simulink library "xbsIndex_r4"  (Simulink 7.1)
PreLoadFcn:
  | warning('off','MATLAB:mex:deprecatedExtension');xlmeta;com.xilinx.sysgen.util.StrategyUtil.loadAllStrategyNames();
values from neighbouring files (symbols this model uses):
  a = xpath.evaluate('//pre:DocumentInfo/pre:Document',x,javax.xml.xpath.XPathConstants.NODESET)    [xlDoc.m]
  n = xpath.evaluate(['//pre:DocumentInfo/pre:Document[@title="'  title                            '"]'],root_elem,javax.xml.xpath.XPathConstants.NODE)    [xlDoc.m]
undefined symbols (not defined in the file or in its folder): gcbh, sim_pause, simulink_period, xlBlockLoadCallback, xlipgetpartsetting, xlRegisterHandles, xlUpdateSgTokenIconStats
libraries: xbsIndex_r4 x18, xbsCopyrightNotice_r4 x1, simulink x1
(part 1 of 9)
settings Model: Tag=SysGenIndex  Creator=sysgengroup  LastModifiedBy=sysgengroup

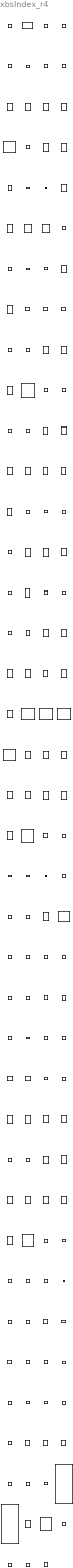
== system xbsIndex_r4 ==
  note: Xilinx Blockset v
      | (c) 2011 Xilinx, Inc.
      |
      | Library Index
  " System Generator" : Subsystem  Tag=genX  LoadFcn=xlUpdateSgTokenIconStats(gcbh);xlBlockLoadCallback(gcbh);  mask(Xilinx System Generator Block){infoedit=System Generator, xilinxfamily=Virtex6, part=xc6vsx315t, speed=-3, package=ff1156, synthesis_tool_sgadvanced=, synthesis_tool=XST, clock_wrapper_sgadvanced=, clock_wrapper=Clock Enables, directory=./netlist, proj_type_sgadvanced=, proj_type=Project Navigator, Synth_file_sgadvanced=, Synth_file=XST Defaults, Impl_file_sgadvanced=, Impl_file=ISE Defaults, testbench_sgadvanced=, testbench=off, simulink_period=1, sysclk_period=10, dcm_input_clock_period=10, incr_netlist_sgadvanced=, incr_netlist=off, trim_vbits_sgadvanced=, trim_vbits=Everywhere in SubSystem, dbl_ovrd_sgadvanced=, dbl_ovrd=According to Block Masks, core_generation_sgadvanced=, core_generation=According to Block Masks, run_coregen_sgadvanced=, run_coregen=off, deprecated_control_sgadvanced=, deprecated_control=off, eval_field=0, has_advanced_control=0, sggui_pos=-1,-1,-1,-1, block_type=sysgen, block_version=, sg_icon_stat=50,50,-1,-1,token,white,0,07734,right,,[ ],[ ], sg_mask_display=|, sg_list_contents=, sg_blockgui_xml=}
      mask sg_mask_display=|
      | fprintf('','COMMENT: begin icon graphics');
      | patch([0 50 50 0 0 ],[0 0 50 50 0 ],[1 1 1 ]);
      | patch([1.6375 16.81 27.31 37.81 48.31 27.31 12.1375 1.6375 ],[36.655 36.655 47.155 36.655 47.155 47.155 47.155 36.655 ],[0.933333 0.203922 0.141176 ]);
      | patch([12.1375 27.31 16.81 1.6375 12.1375 ],[26.155 26.155 36.655 36.655 26.155 ],[0.698039 0.0313725 0.219608 ]);
      | patch([1.6375 16.81 27.31 12.1375 1.6375 ],[15.655 15.655 26.155 26.155 15.655 ],[0.933333 0.203922 0.141176 ]);
      | patch([12.1375 48.31 37.81 27.31 16.81 1.6375 12.1375 ],[5.155 5.155 15.655 5.155 15.655 15.655 5.155 ],[0.698039 0.0313725 0.219608 ]);
      | fprintf('','COMMENT: end icon graphics');
      | fprintf('','COMMENT: begin icon text');
      | fprintf('','COMMENT: end icon text');
      mask prompts: infoedit ""; xilinxfamily "Xilinx family"; synthesis_tool_sgadvanced ""; synthesis_tool "Synthesis tool"; clock_wrapper_sgadvanced ""; clock_wrapper "Clock Wrapper"; directory "Target directory"; proj_type_sgadvanced ""; proj_type "Project Type"; Synth_file_sgadvanced ""; Synth_file "Synthesis strategy"; Impl_file_sgadvanced ""; Impl_file "Implementation strategy"; testbench_sgadvanced ""; simulink_period "Simulink period"; sysclk_period "System clock period"; dcm_input_clock_period "DCM input clock period"; incr_netlist_sgadvanced ""; incr_netlist "Incremental netlisting"; trim_vbits_sgadvanced ""; trim_vbits "Trim valid bits"; dbl_ovrd_sgadvanced ""; dbl_ovrd "Override with doubles"; core_generation_sgadvanced ""; core_generation "Generate cores"; run_coregen_sgadvanced ""; run_coregen "Run CoreGen"; deprecated_control_sgadvanced ""; deprecated_control "Show deprecated controls"; eval_field ""; has_advanced_control ""; sggui_pos ""; block_type ""; block_version ""; sg_icon_stat ""; sg_mask_display ""; sg_list_contents ""; sg_blockgui_xml ""
      mask help: System Generator
      mask init:
      | try
      |   tmp_gcb = gcb;
      |   tmp_gcbh = gcbh;
      |   if (strcmp('SysGenIndex',get_param(bdroot(tmp_gcbh),'tag')) && ~isempty(regexp(bdroot(tmp_gcb), '^xbs', 'once')))
      |     return;
      |   end;
      |   xlMungeMaskParams;
      | 
      |   block_type='sysgen';
      | 
      |   serialized_declarations = '{''block_type''=>''String''}';
      |   ptable_ = xlblockprep(get_param(tmp_gcb, 'MaskWSVariables'));
      |   try
      |     xlBlockMoveCallback(tmp_gcbh);
      |   catch 
      |      clear global xl_updateicon_recursion_guard;
      |   end;
      | catch
      |   global dbgsysgen;
      |   if(~isempty(dbgsysgen) && dbgsysgen)
      |     e = regexprep(lasterr, '\n', '\nError: ');
      |     disp(['Error: While running MaskInit code on block ' tmp_gcb ': ' e]);
      |     error(e);
      |   end
      | end
      settings: AttributesFormatString=System\nGenerator  CopyFcn=xlBlockMoveCallback(gcbh);  DeleteFcn=xlSysgenGUI('delete', gcs, gcbh);  ModelCloseFcn=xlSysgenGUI('Close',gcs,gcbh);  PostSaveFcn=xlSysgenGUI('Save')  OpenFcn=xlSysgenGUI('startup',gcs,gcbh);  MoveFcn=xlBlockMoveCallback(gcbh);
      mask Help: eval('');xlDoc('-book','sysgen','-topic','System_Generator');
      mask StyleString: edit,edit,edit,edit,edit,edit,popup(Spectrum|Synplify|Synplify Pro|XST|RDS|Precision),edit,popup(Clock Enables|Clock Generator(DCM)|Expose Clock Ports),edit,edit,popup(Project Navigator|PlanAhead),edit,popup(XST Defaults|PlanAhead Defaults|Rodin Synthesis Defaults),edit,popup(ISE Defaults|Rodin Implementation Defaults),edit,checkbox,edit,edit,edit,edit,checkbox,edit,popup(According to Block Masks|Everywhere in SubSystem|No Where in SubSystem),edit,popup(According to Block Masks|Everywhere in SubSystem|No Where in SubSystem),edit,popup(According to Block Masks|Everywhere Available|Not Needed - Already Generated),edit,checkbox,edit,checkbox,edit,edit,edit,edit,edit,edit,edit,edit,edit
      mask Display:
      | fprintf('','COMMENT: begin icon graphics');
      | patch([0 50 50 0 0 ],[0 0 50 50 0 ],[1 1 1 ]);
      | patch([1.6375 16.81 27.31 37.81 48.31 27.31 12.1375 1.6375 ],[36.655 36.655 47.155 36.655 47.155 47.155 47.155 36.655 ],[0.933333 0.203922 0.141176 ]);
      | patch([12.1375 27.31 16.81 1.6375 12.1375 ],[26.155 26.155 36.655 36.655 26.155 ],[0.698039 0.0313725 0.219608 ]);
      | patch([1.6375 16.81 27.31 12.1375 1.6375 ],[15.655 15.655 26.155 26.155 15.655 ],[0.933333 0.203922 0.141176 ]);
      | patch([12.1375 48.31 37.81 27.31 16.81 1.6375 12.1375 ],[5.155 5.155 15.655 5.155 15.655 15.655 5.155 ],[0.698039 0.0313725 0.219608 ]);
      | fprintf('','COMMENT: end icon graphics');
      | fprintf('','COMMENT: begin icon text');
      | fprintf('','COMMENT: end icon text');
  AXI FIFO : S-Function  LoadFcn=xlBlockLoadCallback(gcbh);  FunctionName=sysgen  Parameters=ptable_  EnableBusSupport=off  mask(Xilinx AXI FIFO Block Block){input_depth_axis_sgadvanced=, input_depth_axis=1K, actual_fifo_depth_label=1026, enable_tdata_sgadvanced=, enable_tdata=on, enable_tdest_sgadvanced=, enable_tdest=off, enable_tstrb_sgadvanced=, enable_tstrb=off, enable_tready_sgadvanced=, enable_tready=on, enable_tid_sgadvanced=, enable_tid=off, enable_tuser_sgadvanced=, enable_tuser=off, enable_tkeep_sgadvanced=, enable_tkeep=off, enable_tlast_sgadvanced=, enable_tlast=off, has_aresetn_sgadvanced=, has_aresetn=off, underflow_flag_axi_sgadvanced=, underflow_flag_axi=off, underflow_sense_axi_sgadvanced=, underflow_sense_axi=Active High, overflow_flag_axi_sgadvanced=, overflow_flag_axi=off, overflow_sense_axi_sgadvanced=, overflow_sense_axi=Active High, enable_data_counts_axis_sgadvanced=, enable_data_counts_axis=off, fifo_implementation_type_axis_sgadvanced=, fifo_implementation_type_axis=Common Clock Block RAM, trim_axipin_name=on, xlcconfig=, programmable_full_type_axis=Full, full_threshold_assert_value_axis=0, programmable_empty_type_axis=Empty, empty_threshold_assert_value_axis=1022, has_advanced_control=0, sggui_pos=-1,-1,-1,-1, block_type=axi_fifo, block_version=, sg_icon_stat=200,114,3,3,white,blue,0,6408c73b,right,,[2 3 3 ],[2 2 3 ], sg_mask_display=|, sg_list_contents=, sg_blockgui_xml=}
      mask sg_mask_display=|
      | fprintf('','COMMENT: begin icon graphics');
      | patch([0 0 4 4 ],[111 83 83 111 ],[5.466667e-001 5.800000e-001 6.400000e-001 ]);
      | patch([0 0 4 4 ],[71 3 3 71 ],[3.233333e-001 3.400000e-001 3.700000e-001 ]);
      | patch([196 196 200 200 ],[111 43 43 111 ],[5.466667e-001 5.800000e-001 6.400000e-001 ]);
      | patch([196 196 200 200 ],[31 3 3 31 ],[3.233333e-001 3.400000e-001 3.700000e-001 ]);
      | patch([4 195 195 4 4 ],[0 0 114 114 0 ],[7.700000e-001 8.200000e-001 9.100000e-001 ]);
      | plot([4 195 195 4 4 ],[0 0 114 114 0 ]);
      |
      |
      | patch([64.4 87.52 103.52 119.52 135.52 103.52 80.4 64.4 ],[74.76 74.76 90.76 74.76 90.76 90.76 90.76 74.76 ],[1 1 1 ]);
      | patch([80.4 103.52 87.52 64.4 80.4 ],[58.76 58.76 74.76 74.76 58.76 ],[0.931 0.946 0.973 ]);
      | patch([64.4 87.52 103.52 80.4 64.4 ],[42.76 42.76 58.76 58.76 42.76 ],[1 1 1 ]);
      | patch([80.4 135.52 119.52 103.52 87.52 64.4 80.4 ],[26.76 26.76 42.76 26.76 42.76 42.76 26.76 ],[0.931 0.946 0.973 ]);
      | fprintf('','COMMENT: end icon graphics');
      | fprintf('','COMMENT: begin icon text');
      | color('black');port_label('input',1,'  tready  ');
      | color('black');port_label('input',2,'  tvalid  ');
      | color('black');port_label('input',3,'  tdata  ');
      | color('black');port_label('output',1,'  tvalid  ');
      | color('black');port_label('output',2,'  tdata  ');
      | color('black');port_label('output',3,'  tready  ');
      | fprintf('','COMMENT: end icon text');
      mask prompts: input_depth_axis_sgadvanced ""; input_depth_axis "FIFO depth"; actual_fifo_depth_label "Actual FIFO depth"; enable_tdata_sgadvanced ""; enable_tdata "TDATA"; enable_tdest_sgadvanced ""; enable_tdest "TDEST"; enable_tstrb_sgadvanced ""; enable_tstrb "TSTRB"; enable_tready_sgadvanced ""; enable_tready "TREADY"; enable_tid_sgadvanced ""; enable_tid "TID"; enable_tuser_sgadvanced ""; enable_tuser "TUSER"; enable_tkeep_sgadvanced ""; enable_tkeep "TKEEP"; enable_tlast_sgadvanced ""; enable_tlast "TLAST"; has_aresetn_sgadvanced ""; has_aresetn "aresetn"; underflow_flag_axi_sgadvanced ""; underflow_flag_axi "Underflow flag"; underflow_sense_axi_sgadvanced ""; underflow_sense_axi "Underflow (Read Error)"; overflow_flag_axi_sgadvanced ""; overflow_flag_axi "Overflow flag"; overflow_sense_axi_sgadvanced ""; overflow_sense_axi "Overflow (Read Error)"; enable_data_counts_axis_sgadvanced ""; enable_data_counts_axis "Provide FIFO occupancy DATA counts"; fifo_implementation_type_axis_sgadvanced ""; fifo_implementation_type_axis "FIFO implementation type"; trim_axipin_name "Display shortened port names"; xlcconfig ""; programmable_full_type_axis ""; full_threshold_assert_value_axis ""; programmable_empty_type_axis ""; empty_threshold_assert_value_axis ""; has_advanced_control ""; sggui_pos ""; block_type ""; block_version ""; sg_icon_stat ""; sg_mask_display ""; sg_list_contents ""; sg_blockgui_xml ""
      mask help: Xilinx AXI FIFO Block
      mask init:
      | try
      |   tmp_gcb = gcb;
      |   tmp_gcbh = gcbh;
      |   if (strcmp('SysGenIndex',get_param(bdroot(tmp_gcbh),'tag')) && ~isempty(regexp(bdroot(tmp_gcb), '^xbs', 'once')))
      |     return;
      |   end;
      |   xlMungeMaskParams;
      |   block_config = 'sysgen_blockset:AXI_FIFO_config';
      | 
      |   block_type='axi_fifo';
      | 
      |   serialized_declarations = '{''actual_fifo_depth_label''=>''Int'',''empty_threshold_assert_value_axis''=>''Int'',''enable_data_counts_axis''=>''Bool'',''enable_tdata''=>''Bool'',''enable_tdest''=>''Bool'',''enable_tid''=>''Bool'',''enable_tkeep''=>''Bool'',''enable_tlast''=>''Bool'',''enable_tready''=>''Bool'',''enable_tstrb''=>''Bool'',''enable_tuser''=>''Bool'',''fifo_implementation_type_axis''=>''String'',''full_threshold_assert_value_axis''=>''Int'',''has_aresetn''=>''Bool'',''input_depth_axis''=>''Int'',''overflow_flag_axi''=>''Bool'',''overflow_sense_axi''=>''String'',''programmable_empty_type_axis''=>''String'',''programmable_full_type_axis''=>''String'',''trim_axipin_name''=>''Int'',''underflow_flag_axi''=>''Bool'',''underflow_sense_axi''=>''String'',''xlcconfig''=>''String'',''block_type''=>''String''}';
      |   ptable_ = xlblockprep(get_param(tmp_gcb, 'MaskWSVariables'));
      |   try
      |     xlBlockMoveCallback(tmp_gcbh);
      |   catch 
      |      clear global xl_updateicon_recursion_guard;
      |   end;
      | catch
      |   global dbgsysgen;
      |   if(~isempty(dbgsysgen) && dbgsysgen)
      |     e = regexprep(lasterr, '\n', '\nError: ');
      |     disp(['Error: While running MaskInit code on block ' tmp_gcb ': ' e]);
      |     error(e);
      |   end
      | end
      settings: CopyFcn=xlBlockMoveCallback(gcbh);  DeleteFcn=xlDestroyGui(gcbh);  ModelCloseFcn=xlDestroyGui(gcbh);  PreSaveFcn=xlBlockPreSaveCallback(gcbh);  PostSaveFcn=xlBlockPostSaveCallback(gcbh);  DestroyFcn=xlDestroyGui(gcbh);  OpenFcn=xlOpenGui(gcbh, 'axi_fifo_gui.xml', @axi_fifo_enablement, @axi_fifo_action)  CloseFcn=xlDestroyGui(gcbh);  MoveFcn=xlBlockMoveCallback(gcbh);
      mask Help: eval('');xlDoc('-book','sysgen','-topic','AXI_FIFO');
      mask StyleString: edit,popup(16|32|64|128|256|512|1K|2K|4K|8K|16K|32K|64K|128K|256K|512K|1M|2M|4M),edit,edit,checkbox,edit,checkbox,edit,checkbox,edit,checkbox,edit,checkbox,edit,checkbox,edit,checkbox,edit,checkbox,edit,checkbox,edit,checkbox,edit,popup(Active High|Active Low),edit,checkbox,edit,popup(Active High|Active Low),edit,checkbox,edit,popup(Common Clock Block RAM|Common Clock Distributed RAM),checkbox,edit,edit,edit,edit,edit,edit,edit,edit,edit,edit,edit,edit,edit
      mask Display:
      | fprintf('','COMMENT: begin icon graphics');
      | patch([0 0 4 4 ],[111 83 83 111 ],[5.466667e-001 5.800000e-001 6.400000e-001 ]);
      | patch([0 0 4 4 ],[71 3 3 71 ],[3.233333e-001 3.400000e-001 3.700000e-001 ]);
      | patch([196 196 200 200 ],[111 43 43 111 ],[5.466667e-001 5.800000e-001 6.400000e-001 ]);
      | patch([196 196 200 200 ],[31 3 3 31 ],[3.233333e-001 3.400000e-001 3.700000e-001 ]);
      | patch([4 195 195 4 4 ],[0 0 114 114 0 ],[7.700000e-001 8.200000e-001 9.100000e-001 ]);
      | plot([4 195 195 4 4 ],[0 0 114 114 0 ]);
      | 
      | 
      | patch([64.4 87.52 103.52 119.52 135.52 103.52 80.4 64.4 ],[74.76 74.76 90.76 74.76 90.76 90.76 90.76 74.76 ],[1 1 1 ]);
      | patch([80.4 103.52 87.52 64.4 80.4 ],[58.76 58.76 74.76 74.76 58.76 ],[0.931 0.946 0.973 ]);
      | patch([64.4 87.52 103.52 80.4 64.4 ],[42.76 42.76 58.76 58.76 42.76 ],[1 1 1 ]);
      | patch([80.4 135.52 119.52 103.52 87.52 64.4 80.4 ],[26.76 26.76 42.76 26.76 42.76 42.76 26.76 ],[0.931 0.946 0.973 ]);
      | fprintf('','COMMENT: end icon graphics');
      | fprintf('','COMMENT: begin icon text');
      | color('black');port_label('input',1,'  tready  ');
      | color('black');port_label('input',2,'  tvalid  ');
      | color('black');port_label('input',3,'  tdata  ');
      | color('black');port_label('output',1,'  tvalid  ');
      | color('black');port_label('output',2,'  tdata  ');
      | color('black');port_label('output',3,'  tready  ');
      | fprintf('','COMMENT: end icon text');
  Accumulator : S-Function  LoadFcn=xlBlockLoadCallback(gcbh);  FunctionName=sysgen  Parameters=ptable_  EnableBusSupport=off  mask(Xilinx Accumulator Block){infoedit=Adder or subtracter-based accumulator.   Output type and binary point position match the input.<br><br>Hardware notes: When "Reinitialize with input 'b' on reset" is selected, the accumulator is forced to run at the system rate even if the input 'b' is running at a slower rate., operation_sgadvanced=, operation=Add, n_bits=8, overflow_sgadvanced=, overflow=Wrap, scale_sgadvanced=, scale=1, rst_sgadvanced=, rst=on, hasbypass_sgadvanced=, hasbypass=off, en_sgadvanced=, en=off, dbl_ovrd_sgadvanced=, dbl_ovrd=off, use_behavioral_HDL_sgadvanced=, use_behavioral_HDL=on, implementation_sgadvanced=, implementation=Fabric, xl_use_area_sgadvanced=, xl_use_area=off, xl_area=[0,0,0,0,0,0,0], has_advanced_control=0, sggui_pos=-1,-1,-1,-1, block_type=accum, block_version=, sg_icon_stat=60,58,2,1,white,blue,0,6949434e,right,,[ ],[ ], sg_mask_display=|, sg_list_contents=, sg_blockgui_xml=}
      mask sg_mask_display=|
      | fprintf('','COMMENT: begin icon graphics');
      | patch([0 60 60 0 0 ],[0 0 58 58 0 ],[0.77 0.82 0.91 ]);
      | plot([0 60 60 0 0 ],[0 0 58 58 0 ]);
      | patch([12.2 23.76 31.76 39.76 47.76 31.76 20.2 12.2 ],[37.88 37.88 45.88 37.88 45.88 45.88 45.88 37.88 ],[1 1 1 ]);
      | patch([20.2 31.76 23.76 12.2 20.2 ],[29.88 29.88 37.88 37.88 29.88 ],[0.931 0.946 0.973 ]);
      | patch([12.2 23.76 31.76 20.2 12.2 ],[21.88 21.88 29.88 29.88 21.88 ],[1 1 1 ]);
      | patch([20.2 47.76 39.76 31.76 23.76 12.2 20.2 ],[13.88 13.88 21.88 13.88 21.88 21.88 13.88 ],[0.931 0.946 0.973 ]);
      | fprintf('','COMMENT: end icon graphics');
      | fprintf('','COMMENT: begin icon text');
      | color('black');port_label('input',1,'b');
      | color('black');port_label('input',2,'rst');
      | color('black');port_label('output',1,'\bf+=b','texmode','on');
      | fprintf('','COMMENT: end icon text');
      mask prompts: infoedit ""; operation_sgadvanced ""; n_bits "Number of bits"; overflow_sgadvanced ""; scale_sgadvanced ""; scale "Feedback scaling"; rst_sgadvanced ""; rst "Provide synchronous reset port"; hasbypass_sgadvanced ""; hasbypass "Reinitialize with input 'b' on reset"; en_sgadvanced ""; en "Provide enable port"; dbl_ovrd_sgadvanced ""; dbl_ovrd "Override with doubles"; use_behavioral_HDL_sgadvanced ""; use_behavioral_HDL "Use behavioral HDL (otherwise use core)"; implementation_sgadvanced ""; implementation "Implement using"; xl_use_area_sgadvanced ""; xl_use_area "Define FPGA area for resource estimation"; xl_area "FPGA area [slices, FFs, BRAMs, LUTs, IOBs, emb. mults, TBUFs]"; has_advanced_control ""; sggui_pos ""; block_type ""; block_version ""; sg_icon_stat ""; sg_mask_display ""; sg_list_contents ""; sg_blockgui_xml ""
      mask help:
      | Adder or subtracter-based accumulator.   Output type and binary point position match the input.
      |
      | Hardware notes: When "Reinitialize with input 'b' on reset" is selected, the accumulator is forced to run at the system rate even if the input 'b' is running at a slower rate.
      mask init:
      | try
      |   tmp_gcb = gcb;
      |   tmp_gcbh = gcbh;
      |   if (strcmp('SysGenIndex',get_param(bdroot(tmp_gcbh),'tag')) && ~isempty(regexp(bdroot(tmp_gcb), '^xbs', 'once')))
      |     return;
      |   end;
      |   xlMungeMaskParams;
      |   block_config = 'sysgen_blockset:Accum_config';
      | 
      |   block_type='accum';
      | 
      |   serialized_declarations = '{''en''=>''Int'',''hasbypass''=>''Int'',''implementation''=>''String'',''n_bits''=>''Int'',''operation''=>''Int'',''overflow''=>''Int'',''rst''=>''Int'',''scale''=>''Int'',''use_behavioral_HDL''=>''Int'',''block_type''=>''String''}';
      |   ptable_ = xlblockprep(get_param(tmp_gcb, 'MaskWSVariables'));
      |   try
      |     xlBlockMoveCallback(tmp_gcbh);
      |   catch 
      |      clear global xl_updateicon_recursion_guard;
      |   end;
      | catch
      |   global dbgsysgen;
      |   if(~isempty(dbgsysgen) && dbgsysgen)
      |     e = regexprep(lasterr, '\n', '\nError: ');
      |     disp(['Error: While running MaskInit code on block ' tmp_gcb ': ' e]);
      |     error(e);
      |   end
      | end
      settings: CopyFcn=xlBlockMoveCallback(gcbh);  DeleteFcn=xlDestroyGui(gcbh);  ModelCloseFcn=xlDestroyGui(gcbh);  PreSaveFcn=xlBlockPreSaveCallback(gcbh);  PostSaveFcn=xlBlockPostSaveCallback(gcbh);  DestroyFcn=xlDestroyGui(gcbh);  OpenFcn=xlOpenGui(gcbh, 'accum_gui.xml', @accumenablement, -1)  CloseFcn=xlDestroyGui(gcbh);  MoveFcn=xlBlockMoveCallback(gcbh);
      mask Help: eval('');xlDoc('-book','sysgen','-topic','Accumulator');
      mask StyleString: edit,edit,popup(Add|Subtract),edit,edit,popup(Wrap|Saturate|Flag as error),edit,popup(1|1/2|1/4|1/8|1/16|1/32|1/64|1/128|1/256),edit,checkbox,edit,checkbox,edit,checkbox,edit,checkbox,edit,checkbox,edit,popup(Fabric|DSP48),edit,checkbox,edit,edit,edit,edit,edit,edit,edit,edit,edit
      mask Display:
      | fprintf('','COMMENT: begin icon graphics');
      | patch([0 60 60 0 0 ],[0 0 58 58 0 ],[0.77 0.82 0.91 ]);
      | plot([0 60 60 0 0 ],[0 0 58 58 0 ]);
      | patch([12.2 23.76 31.76 39.76 47.76 31.76 20.2 12.2 ],[37.88 37.88 45.88 37.88 45.88 45.88 45.88 37.88 ],[1 1 1 ]);
      | patch([20.2 31.76 23.76 12.2 20.2 ],[29.88 29.88 37.88 37.88 29.88 ],[0.931 0.946 0.973 ]);
      | patch([12.2 23.76 31.76 20.2 12.2 ],[21.88 21.88 29.88 29.88 21.88 ],[1 1 1 ]);
      | patch([20.2 47.76 39.76 31.76 23.76 12.2 20.2 ],[13.88 13.88 21.88 13.88 21.88 21.88 13.88 ],[0.931 0.946 0.973 ]);
      | fprintf('','COMMENT: end icon graphics');
      | fprintf('','COMMENT: begin icon text');
      | color('black');port_label('input',1,'b');
      | color('black');port_label('input',2,'rst');
      | color('black');port_label('output',1,'\bf+=b','texmode','on');
      | fprintf('','COMMENT: end icon text');
  AddSub : S-Function  LoadFcn=xlBlockLoadCallback(gcbh);  FunctionName=sysgen  Parameters=ptable_  EnableBusSupport=off  mask(Xilinx Adder/Subtracter Block){mode_sgadvanced=, mode=Addition, use_carryin_sgadvanced=, use_carryin=off, use_carryout_sgadvanced=, use_carryout=off, en_sgadvanced=, en=off, latency=0, precision_sgadvanced=, precision=Full, arith_type_sgadvanced=, arith_type=Unsigned, n_bits=16, bin_pt=14, quantization_sgadvanced=, quantization=Truncate, overflow_sgadvanced=, overflow=Wrap, dbl_ovrd_sgadvanced=, dbl_ovrd=off, use_behavioral_HDL_sgadvanced=, use_behavioral_HDL=off, hw_selection_sgadvanced=, hw_selection=Fabric, pipelined_sgadvanced=, pipelined=off, xl_use_area_sgadvanced=, xl_use_area=off, xl_area=[0,0,0,0,0,0,0], use_rpm=, has_advanced_control=0, sggui_pos=-1,-1,-1,-1, block_type=addsub, block_version=, sg_icon_stat=60,58,2,1,white,blue,0,e139daf6,right,,[ ],[ ], sg_mask_display=|, sg_list_contents=, sg_blockgui_xml=}
      mask sg_mask_display=|
      | fprintf('','COMMENT: begin icon graphics');
      | patch([0 60 60 0 0 ],[0 0 58 58 0 ],[0.77 0.82 0.91 ]);
      | plot([0 60 60 0 0 ],[0 0 58 58 0 ]);
      | patch([12.2 23.76 31.76 39.76 47.76 31.76 20.2 12.2 ],[37.88 37.88 45.88 37.88 45.88 45.88 45.88 37.88 ],[1 1 1 ]);
      | patch([20.2 31.76 23.76 12.2 20.2 ],[29.88 29.88 37.88 37.88 29.88 ],[0.931 0.946 0.973 ]);
      | patch([12.2 23.76 31.76 20.2 12.2 ],[21.88 21.88 29.88 29.88 21.88 ],[1 1 1 ]);
      | patch([20.2 47.76 39.76 31.76 23.76 12.2 20.2 ],[13.88 13.88 21.88 13.88 21.88 21.88 13.88 ],[0.931 0.946 0.973 ]);
      | fprintf('','COMMENT: end icon graphics');
      | fprintf('','COMMENT: begin icon text');
      | color('black');port_label('input',1,'a');
      | color('black');port_label('input',2,'b');
      | color('black');port_label('output',1,'\bf{a + b}','texmode','on');
      | fprintf('','COMMENT: end icon text');
      mask prompts: mode_sgadvanced ""; mode "Operation"; use_carryin_sgadvanced ""; use_carryin "Provide carry-in port"; use_carryout_sgadvanced ""; use_carryout "Provide carry-out port"; en_sgadvanced ""; en "Provide enable port"; precision_sgadvanced ""; arith_type_sgadvanced ""; arith_type "Arithmetic type"; n_bits "Number of bits"; bin_pt "Binary point"; quantization_sgadvanced ""; overflow_sgadvanced ""; dbl_ovrd_sgadvanced ""; dbl_ovrd "Override with doubles"; use_behavioral_HDL_sgadvanced ""; use_behavioral_HDL "Use behavioral HDL (otherwise use core)"; hw_selection_sgadvanced ""; hw_selection "Implement using"; pipelined_sgadvanced ""; pipelined "Pipeline for maximum performance"; xl_use_area_sgadvanced ""; xl_use_area "Define FPGA area for resource estimation"; xl_area "FPGA area [slices, FFs, BRAMs, LUTs, IOBs, emb. mults, TBUFs]"; use_rpm ""; has_advanced_control ""; sggui_pos ""; block_type ""; block_version ""; sg_icon_stat ""; sg_mask_display ""; sg_list_contents ""; sg_blockgui_xml ""
      mask help: Xilinx Adder/Subtracter
      mask init:
      | try
      |   tmp_gcb = gcb;
      |   tmp_gcbh = gcbh;
      |   if (strcmp('SysGenIndex',get_param(bdroot(tmp_gcbh),'tag')) && ~isempty(regexp(bdroot(tmp_gcb), '^xbs', 'once')))
      |     return;
      |   end;
      |   xlMungeMaskParams;
      |   block_config = 'sysgen_blockset:Addsub_config';
      | 
      |   block_type='addsub';
      | 
      |   serialized_declarations = '{''arith_type''=>''Int'',''bin_pt''=>''Int'',''en''=>''Int'',''hw_selection''=>''String'',''latency''=>''Int'',''mode''=>''Int'',''n_bits''=>''Int'',''overflow''=>''Int'',''pipelined''=>''Int'',''precision''=>''Int'',''quantization''=>''Int'',''rst''=>''Int'',''use_behavioral_HDL''=>''Int'',''use_carryin''=>''Int'',''use_carryout''=>''Int'',''use_rpm''=>''String'',''block_type''=>''String''}';
      |   ptable_ = xlblockprep(get_param(tmp_gcb, 'MaskWSVariables'));
      |   try
      |     xlBlockMoveCallback(tmp_gcbh);
      |   catch 
      |      clear global xl_updateicon_recursion_guard;
      |   end;
      | catch
      |   global dbgsysgen;
      |   if(~isempty(dbgsysgen) && dbgsysgen)
      |     e = regexprep(lasterr, '\n', '\nError: ');
      |     disp(['Error: While running MaskInit code on block ' tmp_gcb ': ' e]);
      |     error(e);
      |   end
      | end
      settings: CopyFcn=xlBlockMoveCallback(gcbh);  DeleteFcn=xlDestroyGui(gcbh);  ModelCloseFcn=xlDestroyGui(gcbh);  PreSaveFcn=xlBlockPreSaveCallback(gcbh);  PostSaveFcn=xlBlockPostSaveCallback(gcbh);  DestroyFcn=xlDestroyGui(gcbh);  OpenFcn=xlOpenGui(gcbh, 'addsub_gui.xml', @addsubenablement, -1)  CloseFcn=xlDestroyGui(gcbh);  MoveFcn=xlBlockMoveCallback(gcbh);
      mask Help: eval('');xlDoc('-book','sysgen','-topic','AddSub');
      mask StyleString: edit,popup(Addition|Subtraction|Addition or Subtraction),edit,checkbox,edit,checkbox,edit,checkbox,edit,edit,popup(Full|User Defined),edit,popup(Signed  (2's comp)|Unsigned),edit,edit,edit,popup(Truncate|Round  (unbiased: +/- Inf)),edit,popup(Wrap|Saturate|Flag as error),edit,checkbox,edit,checkbox,edit,popup(Fabric|DSP48),edit,checkbox,edit,checkbox,edit,edit,edit,edit,edit,edit,edit,edit,edit,edit
      mask Display:
      | fprintf('','COMMENT: begin icon graphics');
      | patch([0 60 60 0 0 ],[0 0 58 58 0 ],[0.77 0.82 0.91 ]);
      | plot([0 60 60 0 0 ],[0 0 58 58 0 ]);
      | patch([12.2 23.76 31.76 39.76 47.76 31.76 20.2 12.2 ],[37.88 37.88 45.88 37.88 45.88 45.88 45.88 37.88 ],[1 1 1 ]);
      | patch([20.2 31.76 23.76 12.2 20.2 ],[29.88 29.88 37.88 37.88 29.88 ],[0.931 0.946 0.973 ]);
      | patch([12.2 23.76 31.76 20.2 12.2 ],[21.88 21.88 29.88 29.88 21.88 ],[1 1 1 ]);
      | patch([20.2 47.76 39.76 31.76 23.76 12.2 20.2 ],[13.88 13.88 21.88 13.88 21.88 21.88 13.88 ],[0.931 0.946 0.973 ]);
      | fprintf('','COMMENT: end icon graphics');
      | fprintf('','COMMENT: begin icon text');
      | color('black');port_label('input',1,'a');
      | color('black');port_label('input',2,'b');
      | color('black');port_label('output',1,'\bf{a + b}','texmode','on');
      | fprintf('','COMMENT: end icon text');
  Addressable Shift Register : S-Function  LoadFcn=xlBlockLoadCallback(gcbh);  FunctionName=sysgen  Parameters=ptable_  EnableBusSupport=off  mask(Xilinx Addressable Shift Register Block){infoedit=Delay of configurable length.  Any element in the delay line can be addressed and driven onto the output port.<br><br>Hardware notes: This block is implemented using SRL16s. If Virtex-4 or Spartan-3 device is used, multiple SRLC16s are cascaded together., infer_latency_sgadvanced=, infer_latency=off, depth=2, initVector=[0], en_sgadvanced=, en=off, dbl_ovrd_sgadvanced=, dbl_ovrd=off, use_behavioral_HDL_sgadvanced=, use_behavioral_HDL=off, Optimization_sgadvanced=, Optimization=Resource, xl_use_area_sgadvanced=, xl_use_area=off, xl_area=[0,0,0,0,0,0,0], use_rpm=, xlcconfig=, has_advanced_control=0, sggui_pos=-1,-1,-1,-1, block_type=addrsr, block_version=, sg_icon_stat=60,58,2,1,white,blue,0,a352fb33,right,,[ ],[ ], sg_mask_display=|, sg_list_contents=, sg_blockgui_xml=}
      mask sg_mask_display=|
      | fprintf('','COMMENT: begin icon graphics');
      | patch([0 60 60 0 0 ],[0 0 58 58 0 ],[0.77 0.82 0.91 ]);
      | plot([0 60 60 0 0 ],[0 0 58 58 0 ]);
      | patch([12.2 23.76 31.76 39.76 47.76 31.76 20.2 12.2 ],[37.88 37.88 45.88 37.88 45.88 45.88 45.88 37.88 ],[1 1 1 ]);
      | patch([20.2 31.76 23.76 12.2 20.2 ],[29.88 29.88 37.88 37.88 29.88 ],[0.931 0.946 0.973 ]);
      | patch([12.2 23.76 31.76 20.2 12.2 ],[21.88 21.88 29.88 29.88 21.88 ],[1 1 1 ]);
      | patch([20.2 47.76 39.76 31.76 23.76 12.2 20.2 ],[13.88 13.88 21.88 13.88 21.88 21.88 13.88 ],[0.931 0.946 0.973 ]);
      | fprintf('','COMMENT: end icon graphics');
      | fprintf('','COMMENT: begin icon text');
      | color('black');port_label('input',1,'d');
      | color('black');port_label('input',2,'addr');
      | color('black');port_label('output',1,'q');
      | fprintf('','COMMENT: end icon text');
      mask prompts: infoedit ""; infer_latency_sgadvanced ""; infer_latency "Infer maximum latency (depth) using address port width"; depth "Maximum latency (depth)"; initVector "Initial value vector"; en_sgadvanced ""; en "Provide enable port"; dbl_ovrd_sgadvanced ""; dbl_ovrd "Override with doubles"; use_behavioral_HDL_sgadvanced ""; use_behavioral_HDL "Use behavioral HDL (otherwise use core)"; Optimization_sgadvanced ""; xl_use_area_sgadvanced ""; xl_use_area "Define FPGA area for resource estimation"; xl_area "FPGA area [slices, FFs, BRAMs, LUTs, IOBs, emb. mults, TBUFs]"; use_rpm ""; xlcconfig ""; has_advanced_control ""; sggui_pos ""; block_type ""; block_version ""; sg_icon_stat ""; sg_mask_display ""; sg_list_contents ""; sg_blockgui_xml ""
      mask help:
      | Delay of configurable length.  Any element in the delay line can be addressed and driven onto the output port.
      |
      | Hardware notes: This block is implemented using SRL16s. If Virtex-4 or Spartan-3 device is used, multiple SRLC16s are cascaded together.
      mask init:
      | try
      |   tmp_gcb = gcb;
      |   tmp_gcbh = gcbh;
      |   if (strcmp('SysGenIndex',get_param(bdroot(tmp_gcbh),'tag')) && ~isempty(regexp(bdroot(tmp_gcb), '^xbs', 'once')))
      |     return;
      |   end;
      |   xlMungeMaskParams;
      |   block_config = 'sysgen_blockset:Addrsr_config';
      | 
      |   block_type='addrsr';
      | 
      |   serialized_declarations = '{''Optimization''=>''Int'',''depth''=>''Int'',''en''=>''Int'',''infer_latency''=>''Int'',''initVector''=>''DoubleVector'',''rpm''=>''Int'',''rst''=>''Int'',''use_behavioral_HDL''=>''Int'',''use_rpm''=>''String'',''xlcconfig''=>''String'',''block_type''=>''String''}';
      |   ptable_ = xlblockprep(get_param(tmp_gcb, 'MaskWSVariables'));
      |   try
      |     xlBlockMoveCallback(tmp_gcbh);
      |   catch 
      |      clear global xl_updateicon_recursion_guard;
      |   end;
      | catch
      |   global dbgsysgen;
      |   if(~isempty(dbgsysgen) && dbgsysgen)
      |     e = regexprep(lasterr, '\n', '\nError: ');
      |     disp(['Error: While running MaskInit code on block ' tmp_gcb ': ' e]);
      |     error(e);
      |   end
      | end
      settings: CopyFcn=xlBlockMoveCallback(gcbh);  DeleteFcn=xlDestroyGui(gcbh);  ModelCloseFcn=xlDestroyGui(gcbh);  PreSaveFcn=xlBlockPreSaveCallback(gcbh);  PostSaveFcn=xlBlockPostSaveCallback(gcbh);  DestroyFcn=xlDestroyGui(gcbh);  OpenFcn=xlOpenGui(gcbh, 'addrsr_gui.xml', @addrsrenablement, -1)  CloseFcn=xlDestroyGui(gcbh);  MoveFcn=xlBlockMoveCallback(gcbh);
      mask Help: eval('');xlDoc('-book','sysgen','-topic','Addressable_Shift_Register');
      mask StyleString: edit,edit,checkbox,edit,edit,edit,checkbox,edit,checkbox,edit,checkbox,edit,popup(Resource|Speed),edit,checkbox,edit,edit,edit,edit,edit,edit,edit,edit,edit,edit,edit
      mask Display:
      | fprintf('','COMMENT: begin icon graphics');
      | patch([0 60 60 0 0 ],[0 0 58 58 0 ],[0.77 0.82 0.91 ]);
      | plot([0 60 60 0 0 ],[0 0 58 58 0 ]);
      | patch([12.2 23.76 31.76 39.76 47.76 31.76 20.2 12.2 ],[37.88 37.88 45.88 37.88 45.88 45.88 45.88 37.88 ],[1 1 1 ]);
      | patch([20.2 31.76 23.76 12.2 20.2 ],[29.88 29.88 37.88 37.88 29.88 ],[0.931 0.946 0.973 ]);
      | patch([12.2 23.76 31.76 20.2 12.2 ],[21.88 21.88 29.88 29.88 21.88 ],[1 1 1 ]);
      | patch([20.2 47.76 39.76 31.76 23.76 12.2 20.2 ],[13.88 13.88 21.88 13.88 21.88 21.88 13.88 ],[0.931 0.946 0.973 ]);
      | fprintf('','COMMENT: end icon graphics');
      | fprintf('','COMMENT: begin icon text');
      | color('black');port_label('input',1,'d');
      | color('black');port_label('input',2,'addr');
      | color('black');port_label('output',1,'q');
      | fprintf('','COMMENT: end icon text');
  Assert : S-Function  LoadFcn=xlBlockLoadCallback(gcbh);  FunctionName=sysgen  Parameters=ptable_  EnableBusSupport=off  mask(Xilinx Assert Block){infoedit=Asserts a user-defined sample rate and/or type on a signal.<br><br>Hardware notes: In hardware this block costs nothing., assert_type_sgadvanced=, assert_type=off, type_source_sgadvanced=, type_source=Explicitly, gui_display_data_type=Fixed-point, arith_type_sgadvanced=, arith_type=Signed  (2's comp), n_bits=16, bin_pt=14, preci_type_sgadvanced=, preci_type=Single, exp_width=8, frac_width=24, assert_rate_sgadvanced=, assert_rate=off, rate_source_sgadvanced=, rate_source=Explicitly, period=1, output_port_sgadvanced=, output_port=on, has_advanced_control=0, sggui_pos=-1,-1,-1,-1, block_type=assert, block_version=, sg_icon_stat=60,30,1,1,white,blue,0,9657e937,right,,[ ],[ ], sg_mask_display=|, sg_list_contents=, sg_blockgui_xml=}
      mask sg_mask_display=|
      | fprintf('','COMMENT: begin icon graphics');
      | patch([0 60 60 0 0 ],[0 0 30 30 0 ],[0.77 0.82 0.91 ]);
      | plot([0 60 60 0 0 ],[0 0 30 30 0 ]);
      | patch([21.1 26.88 30.88 34.88 38.88 30.88 25.1 21.1 ],[19.44 19.44 23.44 19.44 23.44 23.44 23.44 19.44 ],[1 1 1 ]);
      | patch([25.1 30.88 26.88 21.1 25.1 ],[15.44 15.44 19.44 19.44 15.44 ],[0.931 0.946 0.973 ]);
      | patch([21.1 26.88 30.88 25.1 21.1 ],[11.44 11.44 15.44 15.44 11.44 ],[1 1 1 ]);
      | patch([25.1 38.88 34.88 30.88 26.88 21.1 25.1 ],[7.44 7.44 11.44 7.44 11.44 11.44 7.44 ],[0.931 0.946 0.973 ]);
      | fprintf('','COMMENT: end icon graphics');
      | fprintf('','COMMENT: begin icon text');
      |
      |
      | color('black');disp('Assert');
      | fprintf('','COMMENT: end icon text');
      mask prompts: infoedit ""; assert_type_sgadvanced ""; assert_type "Assert type"; type_source_sgadvanced ""; type_source "Specify type:"; gui_display_data_type ""; arith_type_sgadvanced ""; arith_type "Arithmetic type"; n_bits "Number of bits"; bin_pt "Binary point"; preci_type_sgadvanced ""; preci_type ""; exp_width "Exponent width"; frac_width "Fraction width"; assert_rate_sgadvanced ""; assert_rate "Assert rate"; rate_source_sgadvanced ""; rate_source "Specify rate:"; period "Sample rate"; output_port_sgadvanced ""; output_port "Provide output port"; has_advanced_control ""; sggui_pos ""; block_type ""; block_version ""; sg_icon_stat ""; sg_mask_display ""; sg_list_contents ""; sg_blockgui_xml ""
      mask help:
      | Asserts a user-defined sample rate and/or type on a signal.
      |
      | Hardware notes: In hardware this block costs nothing.
      mask init:
      | try
      |   tmp_gcb = gcb;
      |   tmp_gcbh = gcbh;
      |   if (strcmp('SysGenIndex',get_param(bdroot(tmp_gcbh),'tag')) && ~isempty(regexp(bdroot(tmp_gcb), '^xbs', 'once')))
      |     return;
      |   end;
      |   xlMungeMaskParams;
      |   block_config = 'sysgen_blockset:assert_config';
      | 
      |   block_type='assert';
      | 
      |   serialized_declarations = '{''arith_type''=>''Int'',''assert_rate''=>''Int'',''assert_type''=>''Int'',''bin_pt''=>''Int'',''exp_width''=>''Int'',''frac_width''=>''Int'',''gui_display_data_type''=>''Int'',''n_bits''=>''Int'',''output_port''=>''Int'',''period''=>''Double'',''preci_type''=>''Int'',''rate_source''=>''Int'',''type_source''=>''Int'',''block_type''=>''String''}';
      |   ptable_ = xlblockprep(get_param(tmp_gcb, 'MaskWSVariables'));
      |   try
      |     xlBlockMoveCallback(tmp_gcbh);
      |   catch 
      |      clear global xl_updateicon_recursion_guard;
      |   end;
      | catch
      |   global dbgsysgen;
      |   if(~isempty(dbgsysgen) && dbgsysgen)
      |     e = regexprep(lasterr, '\n', '\nError: ');
      |     disp(['Error: While running MaskInit code on block ' tmp_gcb ': ' e]);
      |     error(e);
      |   end
      | end
      settings: CopyFcn=xlBlockMoveCallback(gcbh);  DeleteFcn=xlDestroyGui(gcbh);  ModelCloseFcn=xlDestroyGui(gcbh);  PreSaveFcn=xlBlockPreSaveCallback(gcbh);  PostSaveFcn=xlBlockPostSaveCallback(gcbh);  DestroyFcn=xlDestroyGui(gcbh);  OpenFcn=xlOpenGui(gcbh, 'assert_gui.xml', @assertenablement, @assertaction)  CloseFcn=xlDestroyGui(gcbh);  MoveFcn=xlBlockMoveCallback(gcbh);
      mask Help: eval('');xlDoc('-book','sysgen','-topic','Assert');
      mask StyleString: edit,edit,checkbox,edit,popup(Explicitly|Port),popup(Boolean|Fixed-point|Floating-point),edit,popup(Boolean|Signed  (2's comp)|Unsigned|Floating-point),edit,edit,edit,popup(Single|Double|Custom),edit,edit,edit,checkbox,edit,popup(Explicitly|Port),edit,edit,checkbox,edit,edit,edit,edit,edit,edit,edit,edit
      mask Display:
      | fprintf('','COMMENT: begin icon graphics');
      | patch([0 60 60 0 0 ],[0 0 30 30 0 ],[0.77 0.82 0.91 ]);
      | plot([0 60 60 0 0 ],[0 0 30 30 0 ]);
      | patch([21.1 26.88 30.88 34.88 38.88 30.88 25.1 21.1 ],[19.44 19.44 23.44 19.44 23.44 23.44 23.44 19.44 ],[1 1 1 ]);
      | patch([25.1 30.88 26.88 21.1 25.1 ],[15.44 15.44 19.44 19.44 15.44 ],[0.931 0.946 0.973 ]);
      | patch([21.1 26.88 30.88 25.1 21.1 ],[11.44 11.44 15.44 15.44 11.44 ],[1 1 1 ]);
      | patch([25.1 38.88 34.88 30.88 26.88 21.1 25.1 ],[7.44 7.44 11.44 7.44 11.44 11.44 7.44 ],[0.931 0.946 0.973 ]);
      | fprintf('','COMMENT: end icon graphics');
      | fprintf('','COMMENT: begin icon text');
      | 
      | 
      | color('black');disp('Assert');
      | fprintf('','COMMENT: end icon text');
  BitBasher : S-Function  LoadFcn=xlBlockLoadCallback(gcbh);  FunctionName=sysgen  Parameters=ptable_  EnableBusSupport=off  mask(Xilinx BitBasher Block){infoedit=Allows extraction, concatenation and augmentation of bits, bitexpr=<html><head><meta name="qrichtext" content="1" /></head><body style="font-size:8pt;font-family:MS Shell Dlg"><p>a={b,c[7:3],16'haaf8}</p></body></html>, display_expr_sgadvanced=, display_expr=off, sr_1=1, arith_type1_sgadvanced=, arith_type1=Unsigned, bin_pt1=0, sr_2=2, arith_type2_sgadvanced=, arith_type2=Unsigned, bin_pt2=0, sr_3=3, arith_type3_sgadvanced=, arith_type3=Unsigned, bin_pt3=0, sr_4=4, arith_type4_sgadvanced=, arith_type4=Unsigned, bin_pt4=0, dbl_ovrd_sgadvanced=, dbl_ovrd=off, has_advanced_control=0, sggui_pos=-1,-1,-1,-1, block_type=bitbasher, block_version=, sg_icon_stat=65,60,2,1,white,blue,0,fa88895a,right,,[ ],[ ], sg_mask_display=|, sg_list_contents=, sg_blockgui_xml=}
      mask sg_mask_display=|
      | fprintf('','COMMENT: begin icon graphics');
      | patch([0 65 65 0 0 ],[0 0 60 60 0 ],[0.77 0.82 0.91 ]);
      | plot([0 65 65 0 0 ],[0 0 60 60 0 ]);
      | patch([14.2 25.76 33.76 41.76 49.76 33.76 22.2 14.2 ],[38.88 38.88 46.88 38.88 46.88 46.88 46.88 38.88 ],[1 1 1 ]);
      | patch([22.2 33.76 25.76 14.2 22.2 ],[30.88 30.88 38.88 38.88 30.88 ],[0.931 0.946 0.973 ]);
      | patch([14.2 25.76 33.76 22.2 14.2 ],[22.88 22.88 30.88 30.88 22.88 ],[1 1 1 ]);
      | patch([22.2 49.76 41.76 33.76 25.76 14.2 22.2 ],[14.88 14.88 22.88 14.88 22.88 22.88 14.88 ],[0.931 0.946 0.973 ]);
      | fprintf('','COMMENT: end icon graphics');
      | fprintf('','COMMENT: begin icon text');
      | color('black');port_label('input',1,'b');
      | color('black');port_label('input',2,'c');
      | color('black');port_label('output',1,'a');
      | fprintf('','COMMENT: end icon text');
      mask prompts: infoedit ""; bitexpr "BitBasher Expression"; display_expr_sgadvanced ""; display_expr "Display expression on the block icon"; sr_1 ""; arith_type1_sgadvanced ""; arith_type1 ""; bin_pt1 ""; sr_2 ""; arith_type2_sgadvanced ""; arith_type2 ""; bin_pt2 ""; sr_3 ""; arith_type3_sgadvanced ""; arith_type3 ""; bin_pt3 ""; sr_4 ""; arith_type4_sgadvanced ""; arith_type4 ""; bin_pt4 ""; dbl_ovrd_sgadvanced ""; dbl_ovrd "Override with doubles"; has_advanced_control ""; sggui_pos ""; block_type ""; block_version ""; sg_icon_stat ""; sg_mask_display ""; sg_list_contents ""; sg_blockgui_xml ""
      mask help: Allows extraction, concatenation and augmentation of bits
      mask init:
      | try
      |   tmp_gcb = gcb;
      |   tmp_gcbh = gcbh;
      |   if (strcmp('SysGenIndex',get_param(bdroot(tmp_gcbh),'tag')) && ~isempty(regexp(bdroot(tmp_gcb), '^xbs', 'once')))
      |     return;
      |   end;
      |   xlMungeMaskParams;
      |   block_config = 'sysgen_blockset:BitBasher_config';
      | 
      |   block_type='bitbasher';
      | 
      |   serialized_declarations = '{''arith_type1''=>''Int'',''arith_type2''=>''Int'',''arith_type3''=>''Int'',''arith_type4''=>''Int'',''bin_pt1''=>''Int'',''bin_pt2''=>''Int'',''bin_pt3''=>''Int'',''bin_pt4''=>''Int'',''bitexpr''=>''String'',''chksum''=>''String'',''dbl_ovrd''=>''Int'',''display_expr''=>''Int'',''sim_engine''=>''Int'',''sysgen_root''=>''String'',''block_type''=>''String''}';
      |   xlbitbasher_init();
      |   ptable_ = xlblockprep(get_param(tmp_gcb, 'MaskWSVariables'));
      |   try
      |     xlBlockMoveCallback(tmp_gcbh);
      |   catch 
      |      clear global xl_updateicon_recursion_guard;
      |   end;
      | catch
      |   global dbgsysgen;
      |   if(~isempty(dbgsysgen) && dbgsysgen)
      |     e = regexprep(lasterr, '\n', '\nError: ');
      |     disp(['Error: While running MaskInit code on block ' tmp_gcb ': ' e]);
      |     error(e);
      |   end
      | end
      settings: CopyFcn=xlBlockMoveCallback(gcbh);  DeleteFcn=xlDestroyGui(gcbh);  ModelCloseFcn=xlDestroyGui(gcbh);  PreSaveFcn=xlBlockPreSaveCallback(gcbh);  PostSaveFcn=xlBlockPostSaveCallback(gcbh);  DestroyFcn=xlDestroyGui(gcbh);  OpenFcn=xlOpenGui(gcbh, 'bitbasher_gui.xml', @bitbasherenablement, @bitbasheraction)  CloseFcn=xlDestroyGui(gcbh);  MoveFcn=xlBlockMoveCallback(gcbh);
      mask Help: eval('');xlDoc('-book','sysgen','-topic','BitBasher');
      mask StyleString: edit,edit,edit,checkbox,edit,edit,popup(Unsigned|Signed  (2's comp)),edit,edit,edit,popup(Unsigned|Signed  (2's comp)),edit,edit,edit,popup(Unsigned|Signed  (2's comp)),edit,edit,edit,popup(Unsigned|Signed  (2's comp)),edit,edit,checkbox,edit,edit,edit,edit,edit,edit,edit,edit
      mask Display:
      | fprintf('','COMMENT: begin icon graphics');
      | patch([0 65 65 0 0 ],[0 0 60 60 0 ],[0.77 0.82 0.91 ]);
      | plot([0 65 65 0 0 ],[0 0 60 60 0 ]);
      | patch([14.2 25.76 33.76 41.76 49.76 33.76 22.2 14.2 ],[38.88 38.88 46.88 38.88 46.88 46.88 46.88 38.88 ],[1 1 1 ]);
      | patch([22.2 33.76 25.76 14.2 22.2 ],[30.88 30.88 38.88 38.88 30.88 ],[0.931 0.946 0.973 ]);
      | patch([14.2 25.76 33.76 22.2 14.2 ],[22.88 22.88 30.88 30.88 22.88 ],[1 1 1 ]);
      | patch([22.2 49.76 41.76 33.76 25.76 14.2 22.2 ],[14.88 14.88 22.88 14.88 22.88 22.88 14.88 ],[0.931 0.946 0.973 ]);
      | fprintf('','COMMENT: end icon graphics');
      | fprintf('','COMMENT: begin icon text');
      | color('black');port_label('input',1,'b');
      | color('black');port_label('input',2,'c');
      | color('black');port_label('output',1,'a');
      | fprintf('','COMMENT: end icon text');
  Black Box : S-Function  LoadFcn=xlBlockLoadCallback(gcbh);  FunctionName=sysgen  Parameters=ptable_  EnableBusSupport=off  mask(Xilinx Black Box Block){infoedit=Incorporates black box HDL and simulation model into a System Generator design.<br><br>You must supply a Black Box with certain information about the HDL component you would like to bring into System Generator. This information is provided through a Matlab function.<br><br>When "Simulation mode" is set to "Inactive", you will typically want to provide a separate simulation model by using a Simulation Multiplexer.<br>When "Simulation mode" is set to "External co-simulator", you must include a ModelSim block in the design., init_code=, sim_method_sgadvanced=, sim_method=Inactive, engine_block=, verbose=off, xl_use_area_sgadvanced=, xl_use_area=off, xl_area=[0,0,0,0,0,0,0], has_advanced_control=0, sggui_pos=-1,-1,-1,-1, block_type=blackbox2, block_version=, sg_icon_stat=55,56,0,0,white,blue,0,efd5b770,right,,[ ],[ ], sg_mask_display=|, sg_list_contents=, sg_blockgui_xml=}
      mask sg_mask_display=|
      | fprintf('','COMMENT: begin icon graphics');
      | patch([0 55 55 0 0 ],[0 0 56 56 0 ],[0.77 0.82 0.91 ]);
      | plot([0 55 55 0 0 ],[0 0 56 56 0 ]);
      | patch([11.425 21.54 28.54 35.54 42.54 28.54 18.425 11.425 ],[35.77 35.77 42.77 35.77 42.77 42.77 42.77 35.77 ],[1 1 1 ]);
      | patch([18.425 28.54 21.54 11.425 18.425 ],[28.77 28.77 35.77 35.77 28.77 ],[0.931 0.946 0.973 ]);
      | patch([11.425 21.54 28.54 18.425 11.425 ],[21.77 21.77 28.77 28.77 21.77 ],[1 1 1 ]);
      | patch([18.425 42.54 35.54 28.54 21.54 11.425 18.425 ],[14.77 14.77 21.77 14.77 21.77 21.77 14.77 ],[0.931 0.946 0.973 ]);
      | fprintf('','COMMENT: end icon graphics');
      | fprintf('','COMMENT: begin icon text');
      |
      | fprintf('','COMMENT: end icon text');
      mask prompts: infoedit ""; init_code "Block configuration m-function"; sim_method_sgadvanced ""; sim_method "Simulation mode"; engine_block "HDL co-simulator to use  (specify helper block by name)"; xl_use_area_sgadvanced ""; xl_use_area "Define FPGA area for resource estimation"; xl_area "FPGA area [slices, FFs, BRAMs, LUTs, IOBs, emb. mults, TBUFs]"; has_advanced_control ""; sggui_pos ""; block_type ""; block_version ""; sg_icon_stat ""; sg_mask_display ""; sg_list_contents ""; sg_blockgui_xml ""
      mask help:
      | Incorporates black box HDL and simulation model into a System Generator design.
      |
      | You must supply a Black Box with certain information about the HDL component you would like to bring into System Generator. This information is provided through a Matlab function.
      |
      | When "Simulation mode" is set to "Inactive", you will typically want to provide a separate simulation model by using a Simulation Multiplexer.
      | When "Simulation mode" is set to "External co-simulator", you must include a ModelSim block in the design.
      mask init:
      | try
      |   tmp_gcb = gcb;
      |   tmp_gcbh = gcbh;
      |   if (strcmp('SysGenIndex',get_param(bdroot(tmp_gcbh),'tag')) && ~isempty(regexp(bdroot(tmp_gcb), '^xbs', 'once')))
      |     return;
      |   end;
      |   xlMungeMaskParams;
      |   block_config = 'sysgen_blockset:black_box_config';
      | 
      |   block_type='blackbox2';
      | 
      |   serialized_declarations = '{''engineWorkDir''=>''String'',''engine_block''=>''String'',''engine_handle''=>''Double'',''init_code''=>''String'',''mdlPath''=>''String'',''sim_method''=>''Int'',''srcPath''=>''String'',''validEngineBlock''=>''Int'',''verbose''=>''Bool'',''block_type''=>''String''}';
      |   xlblackbox2_init();
      |   ptable_ = xlblockprep(get_param(tmp_gcb, 'MaskWSVariables'));
      |   try
      |     xlBlockMoveCallback(tmp_gcbh);
      |   catch 
      |      clear global xl_updateicon_recursion_guard;
      |   end;
      | catch
      |   global dbgsysgen;
      |   if(~isempty(dbgsysgen) && dbgsysgen)
      |     e = regexprep(lasterr, '\n', '\nError: ');
      |     disp(['Error: While running MaskInit code on block ' tmp_gcb ': ' e]);
      |     error(e);
      |   end
      | end
      settings: CopyFcn=xlBlockMoveCallback(gcbh);;xlbbCopyCallback;  DeleteFcn=xlDestroyGui(gcbh);  ModelCloseFcn=xlDestroyGui(gcbh);  PreSaveFcn=xlBlockPreSaveCallback(gcbh);  PostSaveFcn=xlBlockPostSaveCallback(gcbh);  DestroyFcn=xlDestroyGui(gcbh);  OpenFcn=xlOpenGui(gcbh, 'blackbox2_gui.xml', @blackbox2enablement, -1)  CloseFcn=xlDestroyGui(gcbh);  MoveFcn=xlBlockMoveCallback(gcbh);
      mask Help: eval('');xlDoc('-book','sysgen','-topic','Black_Box');
      mask StyleString: edit,edit,edit,popup(Inactive|ISE Simulator|External co-simulator),edit,checkbox,edit,checkbox,edit,edit,edit,edit,edit,edit,edit,edit,edit
      mask Display:
      | fprintf('','COMMENT: begin icon graphics');
      | patch([0 55 55 0 0 ],[0 0 56 56 0 ],[0.77 0.82 0.91 ]);
      | plot([0 55 55 0 0 ],[0 0 56 56 0 ]);
      | patch([11.425 21.54 28.54 35.54 42.54 28.54 18.425 11.425 ],[35.77 35.77 42.77 35.77 42.77 42.77 42.77 35.77 ],[1 1 1 ]);
      | patch([18.425 28.54 21.54 11.425 18.425 ],[28.77 28.77 35.77 35.77 28.77 ],[0.931 0.946 0.973 ]);
      | patch([11.425 21.54 28.54 18.425 11.425 ],[21.77 21.77 28.77 28.77 21.77 ],[1 1 1 ]);
      | patch([18.425 42.54 35.54 28.54 21.54 11.425 18.425 ],[14.77 14.77 21.77 14.77 21.77 21.77 14.77 ],[0.931 0.946 0.973 ]);
      | fprintf('','COMMENT: end icon graphics');
      | fprintf('','COMMENT: begin icon text');
      | 
      | fprintf('','COMMENT: end icon text');
  "CIC Compiler 1.1 " : S-Function  LoadFcn=xlBlockLoadCallback(gcbh);  FunctionName=sysgen  Parameters=ptable_  EnableBusSupport=off  mask(Xilinx CIC Compiler 1.1 Block){infoedit=Provides the ability to design and implement Cascaded Integrator-Comb (CIC) filters for a variety of Xilinx FPGA devices.<br><br>Hardware  notes: Optional mapping to DSP48/E/A primitives., filter_type=Interpolation, number_of_stages=3, differential_delay=1, number_of_channels=1, input_data_width=18, output_data_width=18, sample_rate_changes=Fixed, fixed_or_initial_rate=4, minimum_rate=4, maximum_rate=4, ce=off, sclr=off, use_xtreme_dsp_slice=off, xl_use_area=off, xl_area=[0,0,0,0,0,0,0], ip_name=CIC Compiler, ip_version=1.1, dsptool_ready=true, structural_sim=true, has_advanced_control=0, sggui_pos=-1,-1,-1,-1, block_type=cic_compiler_v1_0, block_version=, sg_icon_stat=95,142,-1,-1,white,blue,0,07734,right,,[ ],[ ], sg_mask_display=|, sg_list_contents=, sg_blockgui_xml=}
      mask sg_mask_display=|
      | fprintf('','COMMENT: begin icon graphics');
      | patch([0 95 95 0 0 ],[0 0 142 142 0 ],[0.77 0.82 0.91 ]);
      | plot([0 95 95 0 0 ],[0 0 142 142 0 ]);
      | patch([18.075 36.86 49.86 62.86 75.86 49.86 31.075 18.075 ],[85.43 85.43 98.43 85.43 98.43 98.43 98.43 85.43 ],[1 1 1 ]);
      | patch([31.075 49.86 36.86 18.075 31.075 ],[72.43 72.43 85.43 85.43 72.43 ],[0.931 0.946 0.973 ]);
      | patch([18.075 36.86 49.86 31.075 18.075 ],[59.43 59.43 72.43 72.43 59.43 ],[1 1 1 ]);
      | patch([31.075 75.86 62.86 49.86 36.86 18.075 31.075 ],[46.43 46.43 59.43 46.43 59.43 59.43 46.43 ],[0.931 0.946 0.973 ]);
      | fprintf('','COMMENT: end icon graphics');
      | fprintf('','COMMENT: begin icon text');
      | fprintf('','COMMENT: end icon text');
      mask prompts: infoedit ""; filter_type "Filter type"; number_of_stages "Number of stages"; differential_delay "Differential delay"; number_of_channels "Number of channels"; input_data_width "Input data width"; output_data_width "Output data width"; sample_rate_changes "Sample rate changes"; fixed_or_initial_rate "Fixed or initial rate (ir)"; minimum_rate "Minimum rate (Range: 4..ir)"; maximum_rate "Maximum rate (Range: ir..8192)"; use_xtreme_dsp_slice "Use Xtreme DSP slice"; xl_use_area "Define FPGA area for resource estimation"; xl_area "FPGA area [slices, FFs, BRAMs, LUTs, IOBs, emb. mults, TBUFs]"; ip_name ""; ip_version ""; dsptool_ready ""; structural_sim ""; has_advanced_control ""; sggui_pos ""; block_type ""; block_version ""; sg_icon_stat ""; sg_mask_display ""; sg_list_contents ""; sg_blockgui_xml ""
      mask help:
      | Provides the ability to design and implement Cascaded Integrator-Comb (CIC) filters for a variety of Xilinx FPGA devices.
      |
      | Hardware  notes: Optional mapping to DSP48/E/A primitives.
      mask init:
      | try
      |   tmp_gcb = gcb;
      |   tmp_gcbh = gcbh;
      |   if (strcmp('SysGenIndex',get_param(bdroot(tmp_gcbh),'tag')) && ~isempty(regexp(bdroot(tmp_gcb), '^xbs', 'once')))
      |     return;
      |   end;
      |   xlMungeMaskParams;
      |   block_config = 'sysgen_blockset:Removed_config';
      | 
      |   block_type='cic_compiler_v1_0';
      | nport = get_param(gcbh, 'ports');
      | nin = nport(1);
      | nout = nport(2);
      | 
      |   serialized_declarations = '{''ce''=>''Bool'',''differential_delay''=>''String'',''dsptool_ready''=>''Bool'',''filter_type''=>''String'',''fixed_or_initial_rate''=>''Int'',''input_data_width''=>''Int'',''ip_name''=>''String'',''ip_version''=>''String'',''maximum_rate''=>''Int'',''minimum_rate''=>''Int'',''number_of_channels''=>''String'',''number_of_stages''=>''String'',''output_data_width''=>''Int'',''sample_rate_changes''=>''String'',''sclr''=>''Bool'',''structural_sim''=>''Bool'',''use_xtreme_dsp_slice''=>''Bool'',''xl_use_area''=>''Bool'',''block_type''=>''String'',''nin''=>''Double'',''nout''=>''Double''}';
      |   ptable_ = xlblockprep(get_param(tmp_gcb, 'MaskWSVariables'));
      |   try
      |     xlBlockMoveCallback(tmp_gcbh);
      |   catch 
      |      clear global xl_updateicon_recursion_guard;
      |   end;
      | catch
      |   global dbgsysgen;
      |   if(~isempty(dbgsysgen) && dbgsysgen)
      |     e = regexprep(lasterr, '\n', '\nError: ');
      |     disp(['Error: While running MaskInit code on block ' tmp_gcb ': ' e]);
      |     error(e);
      |   end
      | end
      settings: CopyFcn=xlBlockMoveCallback(gcbh);  DeleteFcn=xlDestroyGui(gcbh);  ModelCloseFcn=xlDestroyGui(gcbh);  PreSaveFcn=xlBlockPreSaveCallback(gcbh);  PostSaveFcn=xlBlockPostSaveCallback(gcbh);  DestroyFcn=xlDestroyGui(gcbh);  OpenFcn=xlOpenGui(gcbh, 'cic_compiler_v1_1_gui.xml', @xlremovedenablement, -1)  CloseFcn=xlDestroyGui(gcbh);  MoveFcn=xlBlockMoveCallback(gcbh);
      mask Help: eval('');xlDoc('-book','sysgen','-topic','CIC_Compiler_1_1');
      mask StyleString: edit,popup(Interpolation|Decimation),popup(3|4|5|6),popup(1|2),popup(1|2|3|4|5|6|7|8|9|10|11|12|13|14|15|16),edit,edit,popup(Fixed|Programmable),edit,edit,edit,checkbox,checkbox,checkbox,checkbox,edit,edit,edit,edit,edit,edit,edit,edit,edit,edit,edit,edit,edit
      mask Display:
      | fprintf('','COMMENT: begin icon graphics');
      | patch([0 95 95 0 0 ],[0 0 142 142 0 ],[0.77 0.82 0.91 ]);
      | plot([0 95 95 0 0 ],[0 0 142 142 0 ]);
      | patch([18.075 36.86 49.86 62.86 75.86 49.86 31.075 18.075 ],[85.43 85.43 98.43 85.43 98.43 98.43 98.43 85.43 ],[1 1 1 ]);
      | patch([31.075 49.86 36.86 18.075 31.075 ],[72.43 72.43 85.43 85.43 72.43 ],[0.931 0.946 0.973 ]);
      | patch([18.075 36.86 49.86 31.075 18.075 ],[59.43 59.43 72.43 72.43 59.43 ],[1 1 1 ]);
      | patch([31.075 75.86 62.86 49.86 36.86 18.075 31.075 ],[46.43 46.43 59.43 46.43 59.43 59.43 46.43 ],[0.931 0.946 0.973 ]);
      | fprintf('','COMMENT: end icon graphics');
      | fprintf('','COMMENT: begin icon text');
      | fprintf('','COMMENT: end icon text');
  "CIC Compiler 1.2 " : S-Function  LoadFcn=xlBlockLoadCallback(gcbh);  FunctionName=sysgen  Parameters=ptable_  EnableBusSupport=off  mask(Xilinx CIC Compiler 1.2 Block){infoedit=Provides the ability to design and implement Cascaded Integrator-Comb (CIC) filters for a variety of Xilinx FPGA devices.<br><br>Hardware  notes: Optional mapping to DSP48/E/A primitives., filter_type=Interpolation, number_of_stages=3, differential_delay=1, number_of_channels=1, input_data_width=18, output_data_width=18, sample_rate_changes=Fixed, fixed_or_initial_rate=4, minimum_rate=4, maximum_rate=4, ce=off, sclr=off, use_xtreme_dsp_slice=off, xl_use_area=off, xl_area=[0,0,0,0,0,0,0], ip_name=CIC Compiler, ip_version=1.2, dsptool_ready=true, structural_sim=false, has_advanced_control=0, sggui_pos=-1,-1,-1,-1, block_type=cic_compiler_v1_2, block_version=, sg_icon_stat=95,142,-1,-1,white,blue,0,07734,right,,[ ],[ ], sg_mask_display=|, sg_list_contents=, sg_blockgui_xml=}
      mask sg_mask_display=|
      | fprintf('','COMMENT: begin icon graphics');
      | patch([0 95 95 0 0 ],[0 0 142 142 0 ],[0.77 0.82 0.91 ]);
      | plot([0 95 95 0 0 ],[0 0 142 142 0 ]);
      | patch([18.075 36.86 49.86 62.86 75.86 49.86 31.075 18.075 ],[85.43 85.43 98.43 85.43 98.43 98.43 98.43 85.43 ],[1 1 1 ]);
      | patch([31.075 49.86 36.86 18.075 31.075 ],[72.43 72.43 85.43 85.43 72.43 ],[0.931 0.946 0.973 ]);
      | patch([18.075 36.86 49.86 31.075 18.075 ],[59.43 59.43 72.43 72.43 59.43 ],[1 1 1 ]);
      | patch([31.075 75.86 62.86 49.86 36.86 18.075 31.075 ],[46.43 46.43 59.43 46.43 59.43 59.43 46.43 ],[0.931 0.946 0.973 ]);
      | fprintf('','COMMENT: end icon graphics');
      | fprintf('','COMMENT: begin icon text');
      | fprintf('','COMMENT: end icon text');
      mask prompts: infoedit ""; filter_type "Filter type"; number_of_stages "Number of stages"; differential_delay "Differential delay"; number_of_channels "Number of channels"; input_data_width "Input data width"; output_data_width "Output data width"; sample_rate_changes "Sample rate changes"; fixed_or_initial_rate "Fixed or initial rate (ir)"; minimum_rate "Minimum rate (Range: 4..ir)"; maximum_rate "Maximum rate (Range: ir..8192)"; use_xtreme_dsp_slice "Use Xtreme DSP slice"; xl_use_area "Define FPGA area for resource estimation"; xl_area "FPGA area [slices, FFs, BRAMs, LUTs, IOBs, emb. mults, TBUFs]"; ip_name ""; ip_version ""; dsptool_ready ""; structural_sim ""; has_advanced_control ""; sggui_pos ""; block_type ""; block_version ""; sg_icon_stat ""; sg_mask_display ""; sg_list_contents ""; sg_blockgui_xml ""
      mask help:
      | Provides the ability to design and implement Cascaded Integrator-Comb (CIC) filters for a variety of Xilinx FPGA devices.
      |
      | Hardware  notes: Optional mapping to DSP48/E/A primitives.
      mask init:
      | try
      |   tmp_gcb = gcb;
      |   tmp_gcbh = gcbh;
      |   if (strcmp('SysGenIndex',get_param(bdroot(tmp_gcbh),'tag')) && ~isempty(regexp(bdroot(tmp_gcb), '^xbs', 'once')))
      |     return;
      |   end;
      |   xlMungeMaskParams;
      |   block_config = 'sysgen_blockset:Removed_config';
      | 
      |   block_type='cic_compiler_v1_2';
      | nport = get_param(gcbh, 'ports');
      | nin = nport(1);
      | nout = nport(2);
      | 
      |   serialized_declarations = '{''ce''=>''Bool'',''differential_delay''=>''String'',''dsptool_ready''=>''Bool'',''filter_type''=>''String'',''fixed_or_initial_rate''=>''Int'',''input_data_width''=>''Int'',''ip_name''=>''String'',''ip_version''=>''String'',''maximum_rate''=>''Int'',''minimum_rate''=>''Int'',''number_of_channels''=>''String'',''number_of_stages''=>''String'',''output_data_width''=>''Int'',''sample_rate_changes''=>''String'',''sclr''=>''Bool'',''structural_sim''=>''Bool'',''use_xtreme_dsp_slice''=>''Bool'',''xl_use_area''=>''Bool'',''block_type''=>''String'',''nin''=>''Double'',''nout''=>''Double''}';
      |   ptable_ = xlblockprep(get_param(tmp_gcb, 'MaskWSVariables'));
      |   try
      |     xlBlockMoveCallback(tmp_gcbh);
      |   catch 
      |      clear global xl_updateicon_recursion_guard;
      |   end;
      | catch
      |   global dbgsysgen;
      |   if(~isempty(dbgsysgen) && dbgsysgen)
      |     e = regexprep(lasterr, '\n', '\nError: ');
      |     disp(['Error: While running MaskInit code on block ' tmp_gcb ': ' e]);
      |     error(e);
      |   end
      | end
      settings: CopyFcn=xlBlockMoveCallback(gcbh);  DeleteFcn=xlDestroyGui(gcbh);  ModelCloseFcn=xlDestroyGui(gcbh);  PreSaveFcn=xlBlockPreSaveCallback(gcbh);  PostSaveFcn=xlBlockPostSaveCallback(gcbh);  DestroyFcn=xlDestroyGui(gcbh);  OpenFcn=xlOpenGui(gcbh, 'cic_compiler_v1_2_gui.xml', @xlremovedenablement, -1)  CloseFcn=xlDestroyGui(gcbh);  MoveFcn=xlBlockMoveCallback(gcbh);
      mask Help: eval('');xlDoc('-book','sysgen','-topic','CIC_Compiler_1_2');
      mask StyleString: edit,popup(Interpolation|Decimation),popup(3|4|5|6),popup(1|2),popup(1|2|3|4|5|6|7|8|9|10|11|12|13|14|15|16),edit,edit,popup(Fixed|Programmable),edit,edit,edit,checkbox,checkbox,checkbox,checkbox,edit,edit,edit,edit,edit,edit,edit,edit,edit,edit,edit,edit,edit
      mask Display:
      | fprintf('','COMMENT: begin icon graphics');
      | patch([0 95 95 0 0 ],[0 0 142 142 0 ],[0.77 0.82 0.91 ]);
      | plot([0 95 95 0 0 ],[0 0 142 142 0 ]);
      | patch([18.075 36.86 49.86 62.86 75.86 49.86 31.075 18.075 ],[85.43 85.43 98.43 85.43 98.43 98.43 98.43 85.43 ],[1 1 1 ]);
      | patch([31.075 49.86 36.86 18.075 31.075 ],[72.43 72.43 85.43 85.43 72.43 ],[0.931 0.946 0.973 ]);
      | patch([18.075 36.86 49.86 31.075 18.075 ],[59.43 59.43 72.43 72.43 59.43 ],[1 1 1 ]);
      | patch([31.075 75.86 62.86 49.86 36.86 18.075 31.075 ],[46.43 46.43 59.43 46.43 59.43 59.43 46.43 ],[0.931 0.946 0.973 ]);
      | fprintf('','COMMENT: end icon graphics');
      | fprintf('','COMMENT: begin icon text');
      | fprintf('','COMMENT: end icon text');
  "CIC Compiler 1.3 " : S-Function  LoadFcn=xlBlockLoadCallback(gcbh);  FunctionName=sysgen  Parameters=ptable_  EnableBusSupport=off  mask(Xilinx CIC Compiler 1.3 Block){filter_type=Interpolation, number_of_stages=3, differential_delay=1, number_of_channels=1, sample_rate_changes=Fixed, fixed_or_initial_rate=4, minimum_rate=4, maximum_rate=4, ratespecification=Maximum_Possible, sampleperiod=4, hardwareoversamplingrate=1, quantization=Full_Precision, output_data_width=18, use_xtreme_dsp_slice=off, use_streaming_interface=on, sclr=off, ce=off, xl_use_area=off, xl_area=[0,0,0,0,0,0,0], gui_behaviour=Sysgen, input_data_width=18, ip_name=CIC Compiler, ip_version=1.3, dsptool_ready=true, wrapper_available=true, port_translation_map={ 'ce' => 'en', 'sclr' => 'rst' }, ipcore_xco_need_fpga_part=true, ipcore_fpga_part=xlipgetpartsetting(gcb, {'virtex4', 'xc4vsx35', '-10', 'ff668'}), ipcore_verbose=false, has_advanced_control=0, sggui_pos=-1,-1,-1,-1, block_type=cic_compiler_v1_3, block_version=, sg_icon_stat=95,142,1,3,white,blue,0,671da946,right,,[ ],[ ], sg_mask_display=|, sg_list_contents=, sg_blockgui_xml=}
      mask sg_mask_display=|
      | fprintf('','COMMENT: begin icon graphics');
      | patch([0 95 95 0 0 ],[0 0 142 142 0 ],[0.77 0.82 0.91 ]);
      | plot([0 95 95 0 0 ],[0 0 142 142 0 ]);
      | patch([18.075 36.86 49.86 62.86 75.86 49.86 31.075 18.075 ],[85.43 85.43 98.43 85.43 98.43 98.43 98.43 85.43 ],[1 1 1 ]);
      | patch([31.075 49.86 36.86 18.075 31.075 ],[72.43 72.43 85.43 85.43 72.43 ],[0.931 0.946 0.973 ]);
      | patch([18.075 36.86 49.86 31.075 18.075 ],[59.43 59.43 72.43 72.43 59.43 ],[1 1 1 ]);
      | patch([31.075 75.86 62.86 49.86 36.86 18.075 31.075 ],[46.43 46.43 59.43 46.43 59.43 59.43 46.43 ],[0.931 0.946 0.973 ]);
      | fprintf('','COMMENT: end icon graphics');
      | fprintf('','COMMENT: begin icon text');
      | color('black');port_label('input',1,'din');
      | color('black');port_label('output',1,'dout');
      | color('black');port_label('output',2,'rfd');
      | color('black');port_label('output',3,'rdy');
      | fprintf('','COMMENT: end icon text');
      mask prompts: filter_type "Filter Type"; number_of_stages "Number of Stages"; differential_delay "Differential Delay"; number_of_channels "Number of Channels"; sample_rate_changes ""; fixed_or_initial_rate "Fixed or Initial Rate"; minimum_rate "Minimum Rate"; maximum_rate "Maximum Rate"; ratespecification "Select format :"; sampleperiod "Sample period :"; hardwareoversamplingrate "Hardware Oversampling Rate :"; output_data_width "Output Data Width"; use_xtreme_dsp_slice "Use Xtreme DSP Slice"; use_streaming_interface "Use Streaming Interface"; sclr "rst"; ce "en"; xl_use_area "Define FPGA area for resource estimation"; xl_area "FPGA area [slices, FFs, BRAMs, LUTs, IOBs, emb. mults, TBUFs]"; gui_behaviour ""; input_data_width ""; ip_name ""; ip_version ""; dsptool_ready ""; wrapper_available ""; port_translation_map ""; ipcore_xco_need_fpga_part ""; ipcore_fpga_part ""; ipcore_verbose ""; has_advanced_control ""; sggui_pos ""; block_type ""; block_version ""; sg_icon_stat ""; sg_mask_display ""; sg_list_contents ""; sg_blockgui_xml ""
      mask help: Xilinx CIC Compiler 1.3
      mask init:
      | try
      |   tmp_gcb = gcb;
      |   tmp_gcbh = gcbh;
      |   if (strcmp('SysGenIndex',get_param(bdroot(tmp_gcbh),'tag')) && ~isempty(regexp(bdroot(tmp_gcb), '^xbs', 'once')))
      |     return;
      |   end;
      |   xlMungeMaskParams;
      |   block_config = 'sysgen:coregenimport_config';
      | 
      |   block_type='cic_compiler_v1_3';
      | 
      |   serialized_declarations = '{''ce''=>''Bool'',''differential_delay''=>''String'',''dsptool_ready''=>''Bool'',''filter_type''=>''String'',''fixed_or_initial_rate''=>''Int'',''gui_behaviour''=>''String'',''hardwareoversamplingrate''=>''Int'',''input_data_width''=>''Int'',''ip_name''=>''String'',''ip_version''=>''String'',''ipcore_fpga_part''=>''StringVector'',''ipcore_verbose''=>''Bool'',''ipcore_xco_need_fpga_part''=>''Bool'',''maximum_rate''=>''Int'',''minimum_rate''=>''Int'',''number_of_channels''=>''String'',''number_of_stages''=>''String'',''output_data_width''=>''Int'',''port_translation_map''=>''String'',''quantization''=>''String'',''ratespecification''=>''String'',''sample_rate_changes''=>''String'',''sampleperiod''=>''Int'',''sclr''=>''Bool'',''use_streaming_interface''=>''Bool'',''use_xtreme_dsp_slice''=>''Bool'',''wrapper_available''=>''Bool'',''xl_use_area''=>''Bool'',''block_type''=>''String''}';
      |   ptable_ = xlblockprep(get_param(tmp_gcb, 'MaskWSVariables'));
      |   try
      |     xlBlockMoveCallback(tmp_gcbh);
      |   catch 
      |      clear global xl_updateicon_recursion_guard;
      |   end;
      | catch
      |   global dbgsysgen;
      |   if(~isempty(dbgsysgen) && dbgsysgen)
      |     e = regexprep(lasterr, '\n', '\nError: ');
      |     disp(['Error: While running MaskInit code on block ' tmp_gcb ': ' e]);
      |     error(e);
      |   end
      | end
      settings: CopyFcn=xlBlockMoveCallback(gcbh);  DeleteFcn=xlDestroyGui(gcbh);  ModelCloseFcn=xlDestroyGui(gcbh);  PreSaveFcn=xlBlockPreSaveCallback(gcbh);  PostSaveFcn=xlBlockPostSaveCallback(gcbh);  DestroyFcn=xlDestroyGui(gcbh);  OpenFcn=xlOpenGui(gcbh, 'cic_compiler_v1_3_gui.xml', @xlipmagiccallback, @xlipmagicaction)  CloseFcn=xlDestroyGui(gcbh);  MoveFcn=xlBlockMoveCallback(gcbh);
      mask Help: eval('');xlDoc('-book','sysgen','-topic','CIC_Compiler_1_3');
      mask StyleString: popup(Interpolation|Decimation),popup(3|4|5|6),popup(1|2),popup(1|2|3|4|5|6|7|8|9|10|11|12|13|14|15|16),popup(Fixed|Programmable),edit,edit,edit,popup(Maximum_Possible|Sample_Period|Hardware_Oversampling_Rate),edit,edit,popup(Full_Precision|Truncation),edit,checkbox,checkbox,checkbox,checkbox,checkbox,edit,edit,edit,edit,edit,edit,edit,edit,edit,edit,edit,edit,edit,edit,edit,edit,edit,edit,edit
      mask Display:
      | fprintf('','COMMENT: begin icon graphics');
      | patch([0 95 95 0 0 ],[0 0 142 142 0 ],[0.77 0.82 0.91 ]);
      | plot([0 95 95 0 0 ],[0 0 142 142 0 ]);
      | patch([18.075 36.86 49.86 62.86 75.86 49.86 31.075 18.075 ],[85.43 85.43 98.43 85.43 98.43 98.43 98.43 85.43 ],[1 1 1 ]);
      | patch([31.075 49.86 36.86 18.075 31.075 ],[72.43 72.43 85.43 85.43 72.43 ],[0.931 0.946 0.973 ]);
      | patch([18.075 36.86 49.86 31.075 18.075 ],[59.43 59.43 72.43 72.43 59.43 ],[1 1 1 ]);
      | patch([31.075 75.86 62.86 49.86 36.86 18.075 31.075 ],[46.43 46.43 59.43 46.43 59.43 59.43 46.43 ],[0.931 0.946 0.973 ]);
      | fprintf('','COMMENT: end icon graphics');
      | fprintf('','COMMENT: begin icon text');
      | color('black');port_label('input',1,'din');
      | color('black');port_label('output',1,'dout');
      | color('black');port_label('output',2,'rfd');
      | color('black');port_label('output',3,'rdy');
      | fprintf('','COMMENT: end icon text');
  "CIC Compiler 2.0 " : S-Function  LoadFcn=xlBlockLoadCallback(gcbh);  FunctionName=sysgen  Parameters=ptable_  EnableBusSupport=off  mask(Xilinx CIC Compiler 2.0 Block){filter_type=Interpolation, number_of_stages=3, differential_delay=1, number_of_channels=1, sample_rate_changes=Fixed, fixed_or_initial_rate=4, minimum_rate=4, maximum_rate=4, ratespecification=Maximum_Possible, sampleperiod=4, hardwareoversamplingrate=1, quantization=Full_Precision, output_data_width=18, use_xtreme_dsp_slice=on, use_streaming_interface=on, sclr=off, ce=off, xl_use_area=off, xl_area=[0,0,0,0,0,0,0], gui_behaviour=Sysgen, input_data_width=18, ip_name=CIC Compiler, ip_version=2.0, dsptool_ready=true, wrapper_available=true, port_translation_map={ 'ce' => 'en', 'sclr' => 'rst' }, ipcore_xco_need_fpga_part=true, ipcore_fpga_part=xlipgetpartsetting(gcb, {'virtex4', 'xc4vsx35', '-10', 'ff668'}), ipcore_verbose=false, has_advanced_control=0, sggui_pos=-1,-1,-1,-1, block_type=cic_compiler_v2_0, block_version=, sg_icon_stat=95,142,1,3,white,blue,0,671da946,right,,[ ],[ ], sg_mask_display=|, sg_list_contents=, sg_blockgui_xml=}
      mask sg_mask_display=|
      | fprintf('','COMMENT: begin icon graphics');
      | patch([0 95 95 0 0 ],[0 0 142 142 0 ],[0.77 0.82 0.91 ]);
      | plot([0 95 95 0 0 ],[0 0 142 142 0 ]);
      | patch([18.075 36.86 49.86 62.86 75.86 49.86 31.075 18.075 ],[85.43 85.43 98.43 85.43 98.43 98.43 98.43 85.43 ],[1 1 1 ]);
      | patch([31.075 49.86 36.86 18.075 31.075 ],[72.43 72.43 85.43 85.43 72.43 ],[0.931 0.946 0.973 ]);
      | patch([18.075 36.86 49.86 31.075 18.075 ],[59.43 59.43 72.43 72.43 59.43 ],[1 1 1 ]);
      | patch([31.075 75.86 62.86 49.86 36.86 18.075 31.075 ],[46.43 46.43 59.43 46.43 59.43 59.43 46.43 ],[0.931 0.946 0.973 ]);
      | fprintf('','COMMENT: end icon graphics');
      | fprintf('','COMMENT: begin icon text');
      | color('black');port_label('input',1,'din');
      | color('black');port_label('output',1,'dout');
      | color('black');port_label('output',2,'rfd');
      | color('black');port_label('output',3,'rdy');
      | fprintf('','COMMENT: end icon text');
      mask prompts: filter_type "Filter Type"; number_of_stages "Number of Stages"; differential_delay "Differential Delay"; number_of_channels "Number of Channels"; sample_rate_changes ""; fixed_or_initial_rate "Fixed or Initial Rate"; minimum_rate "Minimum Rate"; maximum_rate "Maximum Rate"; ratespecification "Select format :"; sampleperiod "Sample period :"; hardwareoversamplingrate "Hardware Oversampling Rate :"; output_data_width "Output Data Width"; use_xtreme_dsp_slice "Use Xtreme DSP Slice"; use_streaming_interface "Use Streaming Interface"; sclr "rst"; ce "en"; xl_use_area "Define FPGA area for resource estimation"; xl_area "FPGA area [slices, FFs, BRAMs, LUTs, IOBs, emb. mults, TBUFs]"; gui_behaviour ""; input_data_width ""; ip_name ""; ip_version ""; dsptool_ready ""; wrapper_available ""; port_translation_map ""; ipcore_xco_need_fpga_part ""; ipcore_fpga_part ""; ipcore_verbose ""; has_advanced_control ""; sggui_pos ""; block_type ""; block_version ""; sg_icon_stat ""; sg_mask_display ""; sg_list_contents ""; sg_blockgui_xml ""
      mask help: Xilinx CIC Compiler 2.0
      mask init:
      | try
      |   tmp_gcb = gcb;
      |   tmp_gcbh = gcbh;
      |   if (strcmp('SysGenIndex',get_param(bdroot(tmp_gcbh),'tag')) && ~isempty(regexp(bdroot(tmp_gcb), '^xbs', 'once')))
      |     return;
      |   end;
      |   xlMungeMaskParams;
      |   block_config = 'sysgen:coregenimport_config';
      | 
      |   block_type='cic_compiler_v2_0';
      | 
      |   serialized_declarations = '{''ce''=>''Bool'',''differential_delay''=>''String'',''dsptool_ready''=>''Bool'',''filter_type''=>''String'',''fixed_or_initial_rate''=>''Int'',''gui_behaviour''=>''String'',''hardwareoversamplingrate''=>''Int'',''input_data_width''=>''Int'',''ip_name''=>''String'',''ip_version''=>''String'',''ipcore_fpga_part''=>''StringVector'',''ipcore_verbose''=>''Bool'',''ipcore_xco_need_fpga_part''=>''Bool'',''maximum_rate''=>''Int'',''minimum_rate''=>''Int'',''number_of_channels''=>''String'',''number_of_stages''=>''String'',''output_data_width''=>''Int'',''port_translation_map''=>''String'',''quantization''=>''String'',''ratespecification''=>''String'',''sample_rate_changes''=>''String'',''sampleperiod''=>''Int'',''sclr''=>''Bool'',''use_streaming_interface''=>''Bool'',''use_xtreme_dsp_slice''=>''Bool'',''wrapper_available''=>''Bool'',''xl_use_area''=>''Bool'',''block_type''=>''String''}';
      |   ptable_ = xlblockprep(get_param(tmp_gcb, 'MaskWSVariables'));
      |   try
      |     xlBlockMoveCallback(tmp_gcbh);
      |   catch 
      |      clear global xl_updateicon_recursion_guard;
      |   end;
      | catch
      |   global dbgsysgen;
      |   if(~isempty(dbgsysgen) && dbgsysgen)
      |     e = regexprep(lasterr, '\n', '\nError: ');
      |     disp(['Error: While running MaskInit code on block ' tmp_gcb ': ' e]);
      |     error(e);
      |   end
      | end
      settings: CopyFcn=xlBlockMoveCallback(gcbh);  DeleteFcn=xlDestroyGui(gcbh);  ModelCloseFcn=xlDestroyGui(gcbh);  PreSaveFcn=xlBlockPreSaveCallback(gcbh);  PostSaveFcn=xlBlockPostSaveCallback(gcbh);  DestroyFcn=xlDestroyGui(gcbh);  OpenFcn=xlOpenGui(gcbh, 'cic_compiler_v2_0_gui.xml', @xlipmagiccallback_pass_evaluate_params, @xlipmagicaction)  CloseFcn=xlDestroyGui(gcbh);  MoveFcn=xlBlockMoveCallback(gcbh);
      mask Help: eval('');xlDoc('-book','sysgen','-topic','CIC_Compiler_2_0');
      mask StyleString: popup(Interpolation|Decimation),popup(3|4|5|6),popup(1|2),popup(1|2|3|4|5|6|7|8|9|10|11|12|13|14|15|16),popup(Fixed|Programmable),edit,edit,edit,popup(Maximum_Possible|Sample_Period|Hardware_Oversampling_Rate),edit,edit,popup(Full_Precision|Truncation),edit,checkbox,checkbox,checkbox,checkbox,checkbox,edit,edit,edit,edit,edit,edit,edit,edit,edit,edit,edit,edit,edit,edit,edit,edit,edit,edit,edit
      mask Display:
      | fprintf('','COMMENT: begin icon graphics');
      | patch([0 95 95 0 0 ],[0 0 142 142 0 ],[0.77 0.82 0.91 ]);
      | plot([0 95 95 0 0 ],[0 0 142 142 0 ]);
      | patch([18.075 36.86 49.86 62.86 75.86 49.86 31.075 18.075 ],[85.43 85.43 98.43 85.43 98.43 98.43 98.43 85.43 ],[1 1 1 ]);
      | patch([31.075 49.86 36.86 18.075 31.075 ],[72.43 72.43 85.43 85.43 72.43 ],[0.931 0.946 0.973 ]);
      | patch([18.075 36.86 49.86 31.075 18.075 ],[59.43 59.43 72.43 72.43 59.43 ],[1 1 1 ]);
      | patch([31.075 75.86 62.86 49.86 36.86 18.075 31.075 ],[46.43 46.43 59.43 46.43 59.43 59.43 46.43 ],[0.931 0.946 0.973 ]);
      | fprintf('','COMMENT: end icon graphics');
      | fprintf('','COMMENT: begin icon text');
      | color('black');port_label('input',1,'din');
      | color('black');port_label('output',1,'dout');
      | color('black');port_label('output',2,'rfd');
      | color('black');port_label('output',3,'rdy');
      | fprintf('','COMMENT: end icon text');
  "CIC Compiler 3.0 " : S-Function  LoadFcn=xlBlockLoadCallback(gcbh);  FunctionName=sysgen  Parameters=ptable_  EnableBusSupport=off  mask(Xilinx CIC Compiler 3.0 Block){filter_type=Interpolation, number_of_stages=3, differential_delay=1, number_of_channels=1, sample_rate_changes=Fixed, fixed_or_initial_rate=4, minimum_rate=4, maximum_rate=4, ratespecification=Maximum_Possible, sampleperiod=4, hardwareoversamplingrate=1, quantization=Full_Precision, output_data_width=22, use_xtreme_dsp_slice=on, use_streaming_interface=on, has_aclken=off, has_aresetn=off, has_dout_tready=off, xl_use_area=off, xl_area=[0,0,0,0,0,0,0], trim_axipin_name=on, gui_behaviour=Sysgen_GUI, input_data_width=18, ip_name=CIC Compiler, ip_version=3.0, dsptool_ready=true, wrapper_available=true, port_translation_map={ 'aclken' => 'en', 'aresetn' => 'rst' }, ipcore_xco_need_fpga_part=true, ipcore_fpga_part=xlipgetpartsetting(gcb, {'virtex7', 'xc7v1500t', '-2', 'fhg1157'}), ipcore_verbose=false, has_advanced_control=0, sggui_pos=-1,-1,-1,-1, block_type=cic_compiler_v3_0, block_version=, sg_icon_stat=240,206,1,3,white,blue,0,30edc886,right,,[2 ],[2 3 3 ], sg_mask_display=|, sg_list_contents=, sg_blockgui_xml=}
      mask sg_mask_display=|
      | fprintf('','COMMENT: begin icon graphics');
      | patch([0 0 4 4 ],[172 34 34 172 ],[5.466667e-001 5.800000e-001 6.400000e-001 ]);
      | patch([236 236 240 240 ],[197 149 149 197 ],[5.466667e-001 5.800000e-001 6.400000e-001 ]);
      | patch([236 236 240 240 ],[127 9 9 127 ],[3.233333e-001 3.400000e-001 3.700000e-001 ]);
      | patch([4 235 235 4 4 ],[0 0 206 206 0 ],[7.700000e-001 8.200000e-001 9.100000e-001 ]);
      | plot([4 235 235 4 4 ],[0 0 206 206 0 ]);
      |
      |
      | patch([55.475 97.38 126.38 155.38 184.38 126.38 84.475 55.475 ],[135.19 135.19 164.19 135.19 164.19 164.19 164.19 135.19 ],[1 1 1 ]);
      | patch([84.475 126.38 97.38 55.475 84.475 ],[106.19 106.19 135.19 135.19 106.19 ],[0.931 0.946 0.973 ]);
      | patch([55.475 97.38 126.38 84.475 55.475 ],[77.19 77.19 106.19 106.19 77.19 ],[1 1 1 ]);
      | patch([84.475 184.38 155.38 126.38 97.38 55.475 84.475 ],[48.19 48.19 77.19 48.19 77.19 77.19 48.19 ],[0.931 0.946 0.973 ]);
      | fprintf('','COMMENT: end icon graphics');
      | fprintf('','COMMENT: begin icon text');
      | color('black');port_label('input',1,'  data_tdata_data  ');
      | color('black');port_label('output',1,'  data_tready  ');
      | color('black');port_label('output',2,'  data_tvalid  ');
      | color('black');port_label('output',3,'  data_tdata_data  ');
      | fprintf('','COMMENT: end icon text');
      mask prompts: filter_type "Filter Type"; number_of_stages "Number of Stages"; differential_delay "Differential Delay"; number_of_channels "Number of Channels"; sample_rate_changes ""; fixed_or_initial_rate "Fixed or Initial Rate"; minimum_rate "Minimum Rate"; maximum_rate "Maximum Rate"; ratespecification "Select format :"; sampleperiod "Sample period :"; hardwareoversamplingrate "Hardware Oversampling Rate :"; output_data_width "Output Data Width"; use_xtreme_dsp_slice "Use Xtreme DSP Slice"; use_streaming_interface "Use Streaming Interface"; has_aclken "ACLKEN"; has_aresetn "ARESETn"; has_dout_tready "Has TREADY"; xl_use_area "Define FPGA area for resource estimation"; xl_area "FPGA area [slices, FFs, BRAMs, LUTs, IOBs, emb. mults, TBUFs]"; trim_axipin_name "Display shortened port names"; gui_behaviour ""; input_data_width ""; ip_name ""; ip_version ""; dsptool_ready ""; wrapper_available ""; port_translation_map ""; ipcore_xco_need_fpga_part ""; ipcore_fpga_part ""; ipcore_verbose ""; has_advanced_control ""; sggui_pos ""; block_type ""; block_version ""; sg_icon_stat ""; sg_mask_display ""; sg_list_contents ""; sg_blockgui_xml ""
      mask help: Xilinx CIC Compiler 3.0
      mask init:
      | try
      |   tmp_gcb = gcb;
      |   tmp_gcbh = gcbh;
      |   if (strcmp('SysGenIndex',get_param(bdroot(tmp_gcbh),'tag')) && ~isempty(regexp(bdroot(tmp_gcb), '^xbs', 'once')))
      |     return;
      |   end;
      |   xlMungeMaskParams;
      |   block_config = 'sysgen:coregenimport_config';
      | 
      |   block_type='cic_compiler_v3_0';
      | 
      |   serialized_declarations = '{''differential_delay''=>''String'',''dsptool_ready''=>''Bool'',''filter_type''=>''String'',''fixed_or_initial_rate''=>''Int'',''gui_behaviour''=>''String'',''hardwareoversamplingrate''=>''Int'',''has_aclken''=>''Bool'',''has_aresetn''=>''Bool'',''has_dout_tready''=>''Bool'',''input_data_width''=>''Int'',''ip_name''=>''String'',''ip_version''=>''String'',''ipcore_fpga_part''=>''StringVector'',''ipcore_verbose''=>''Bool'',''ipcore_xco_need_fpga_part''=>''Bool'',''maximum_rate''=>''Int'',''minimum_rate''=>''Int'',''number_of_channels''=>''String'',''number_of_stages''=>''String'',''output_data_width''=>''Int'',''port_translation_map''=>''String'',''quantization''=>''String'',''ratespecification''=>''String'',''sample_rate_changes''=>''String'',''sampleperiod''=>''Int'',''trim_axipin_name''=>''Int'',''use_streaming_interface''=>''Bool'',''use_xtreme_dsp_slice''=>''Bool'',''wrapper_available''=>''Bool'',''xl_use_area''=>''Bool'',''block_type''=>''String''}';
      |   ptable_ = xlblockprep(get_param(tmp_gcb, 'MaskWSVariables'));
      |   try
      |     xlBlockMoveCallback(tmp_gcbh);
      |   catch 
      |      clear global xl_updateicon_recursion_guard;
      |   end;
      | catch
      |   global dbgsysgen;
      |   if(~isempty(dbgsysgen) && dbgsysgen)
      |     e = regexprep(lasterr, '\n', '\nError: ');
      |     disp(['Error: While running MaskInit code on block ' tmp_gcb ': ' e]);
      |     error(e);
      |   end
      | end
      settings: CopyFcn=xlBlockMoveCallback(gcbh);  DeleteFcn=xlDestroyGui(gcbh);  ModelCloseFcn=xlDestroyGui(gcbh);  PreSaveFcn=xlBlockPreSaveCallback(gcbh);  PostSaveFcn=xlBlockPostSaveCallback(gcbh);  DestroyFcn=xlDestroyGui(gcbh);  OpenFcn=xlOpenGui(gcbh, 'cic_compiler_v3_0_gui.xml', @xlipmagiccallback_pass_evaluate_params, @xlipmagicaction)  CloseFcn=xlDestroyGui(gcbh);  MoveFcn=xlBlockMoveCallback(gcbh);
      mask Help: eval('');xlDoc('-book','sysgen','-topic','CIC_Compiler_3_0');
      mask StyleString: popup(Interpolation|Decimation),popup(3|4|5|6),popup(1|2),popup(1|2|3|4|5|6|7|8|9|10|11|12|13|14|15|16),popup(Fixed|Programmable),edit,edit,edit,popup(Maximum_Possible|Sample_Period|Hardware_Oversampling_Rate),edit,edit,popup(Full_Precision|Truncation),edit,checkbox,checkbox,checkbox,checkbox,checkbox,checkbox,edit,checkbox,edit,edit,edit,edit,edit,edit,edit,edit,edit,edit,edit,edit,edit,edit,edit,edit,edit,edit
      mask Display:
      | fprintf('','COMMENT: begin icon graphics');
      | patch([0 0 4 4 ],[172 34 34 172 ],[5.466667e-001 5.800000e-001 6.400000e-001 ]);
      | patch([236 236 240 240 ],[197 149 149 197 ],[5.466667e-001 5.800000e-001 6.400000e-001 ]);
      | patch([236 236 240 240 ],[127 9 9 127 ],[3.233333e-001 3.400000e-001 3.700000e-001 ]);
      | patch([4 235 235 4 4 ],[0 0 206 206 0 ],[7.700000e-001 8.200000e-001 9.100000e-001 ]);
      | plot([4 235 235 4 4 ],[0 0 206 206 0 ]);
      | 
      | 
      | patch([55.475 97.38 126.38 155.38 184.38 126.38 84.475 55.475 ],[135.19 135.19 164.19 135.19 164.19 164.19 164.19 135.19 ],[1 1 1 ]);
      | patch([84.475 126.38 97.38 55.475 84.475 ],[106.19 106.19 135.19 135.19 106.19 ],[0.931 0.946 0.973 ]);
      | patch([55.475 97.38 126.38 84.475 55.475 ],[77.19 77.19 106.19 106.19 77.19 ],[1 1 1 ]);
      | patch([84.475 184.38 155.38 126.38 97.38 55.475 84.475 ],[48.19 48.19 77.19 48.19 77.19 77.19 48.19 ],[0.931 0.946 0.973 ]);
      | fprintf('','COMMENT: end icon graphics');
      | fprintf('','COMMENT: begin icon text');
      | color('black');port_label('input',1,'  data_tdata_data  ');
      | color('black');port_label('output',1,'  data_tready  ');
      | color('black');port_label('output',2,'  data_tvalid  ');
      | color('black');port_label('output',3,'  data_tdata_data  ');
      | fprintf('','COMMENT: end icon text');
  CMult : S-Function  LoadFcn=xlBlockLoadCallback(gcbh);  FunctionName=sysgen  Parameters=ptable_  EnableBusSupport=off  mask(Xilinx Constant Multiplier Block){const=1, gui_display_data_type_sgadvanced=, gui_display_data_type=Fixed-point, const_n_bits=16, const_bin_pt=14, float_type_sgadvanced=, float_type=Single, exp_bits=8, fraction_bits=24, en_sgadvanced=, en=off, latency=0, precision_sgadvanced=, precision=Full, arith_type_sgadvanced=, arith_type=Signed  (2's comp), n_bits=16, bin_pt=14, quantization_sgadvanced=, quantization=Truncate, overflow_sgadvanced=, overflow=Wrap, dbl_ovrd_sgadvanced=, dbl_ovrd=off, use_behavioral_HDL_sgadvanced=, use_behavioral_HDL=off, mem_type_sgadvanced=, mem_type=Distributed RAM, pipeline_sgadvanced=, pipeline=off, xl_use_area_sgadvanced=, xl_use_area=off, xl_area=[0,0,0,0,0,0,0], use_rpm=, placement_style=, infoedit=, has_advanced_control=0, sggui_pos=-1,-1,-1,-1, block_type=cmult, block_version=, sg_icon_stat=65,60,1,1,white,blue,2,b841b069,right,,[ ],[ ], sg_mask_display=|, sg_list_contents=, sg_blockgui_xml=}
      mask sg_mask_display=|
      | fprintf('','COMMENT: begin icon graphics');
      | patch([0 65 0 0 ],[0 30 60 0 ],[0.77 0.82 0.91 ]);
      | plot([0 65 0 0 ],[0 30 60 0 ]);
      | patch([5.07 12.006 16.806 21.606 26.406 16.806 9.87 5.07 ],[35.328 35.328 40.128 35.328 40.128 40.128 40.128 35.328 ],[1 1 1 ]);
      | patch([9.87 16.806 12.006 5.07 9.87 ],[30.528 30.528 35.328 35.328 30.528 ],[0.931 0.946 0.973 ]);
      | patch([5.07 12.006 16.806 9.87 5.07 ],[25.728 25.728 30.528 30.528 25.728 ],[1 1 1 ]);
      | patch([9.87 26.406 21.606 16.806 12.006 5.07 9.87 ],[20.928 20.928 25.728 20.928 25.728 25.728 20.928 ],[0.931 0.946 0.973 ]);
      | fprintf('','COMMENT: end icon graphics');
      | fprintf('','COMMENT: begin icon text');
      |
      |
      | color('black');disp('\bf{x 1}','texmode','on');
      | fprintf('','COMMENT: end icon text');
      mask prompts: const "Constant value"; gui_display_data_type_sgadvanced ""; gui_display_data_type ""; const_n_bits "Number of bits"; const_bin_pt "Binary point"; float_type_sgadvanced ""; float_type ""; exp_bits "Exponent width"; fraction_bits "Fraction width"; en_sgadvanced ""; en "Provide enable port"; precision_sgadvanced ""; arith_type_sgadvanced ""; arith_type "Arithmetic type"; n_bits "Number of bits"; bin_pt "Binary point"; quantization_sgadvanced ""; overflow_sgadvanced ""; dbl_ovrd_sgadvanced ""; dbl_ovrd "Override with doubles"; use_behavioral_HDL_sgadvanced ""; use_behavioral_HDL "Use behavioral HDL (otherwise use core)"; mem_type_sgadvanced ""; mem_type "Implement using"; pipeline_sgadvanced ""; pipeline "Test for optimum pipelining"; xl_use_area_sgadvanced ""; xl_use_area "Define FPGA area for resource estimation"; xl_area "FPGA area [slices, FFs, BRAMs, LUTs, IOBs, emb. mults, TBUFs]"; use_rpm ""; placement_style ""; infoedit ""; has_advanced_control ""; sggui_pos ""; block_type ""; block_version ""; sg_icon_stat ""; sg_mask_display ""; sg_list_contents ""; sg_blockgui_xml ""
      mask help: Xilinx Constant Multiplier
      mask init:
      | try
      |   tmp_gcb = gcb;
      |   tmp_gcbh = gcbh;
      |   if (strcmp('SysGenIndex',get_param(bdroot(tmp_gcbh),'tag')) && ~isempty(regexp(bdroot(tmp_gcb), '^xbs', 'once')))
      |     return;
      |   end;
      |   xlMungeMaskParams;
      |   block_config = 'sysgen_blockset:CMult_config';
      | 
      |   block_type='cmult';
      | 
      |   serialized_declarations = '{''arith_type''=>''Int'',''bin_pt''=>''Int'',''const''=>''Double'',''const_bin_pt''=>''Int'',''const_n_bits''=>''Int'',''dbl_ovrd''=>''Int'',''en''=>''Int'',''exp_bits''=>''Int'',''float_type''=>''Int'',''fraction_bits''=>''Int'',''gui_display_data_type''=>''Int'',''latency''=>''Int'',''mem_type''=>''Int'',''n_bits''=>''Int'',''overflow''=>''Int'',''pipeline''=>''Int'',''placement_style''=>''String'',''precision''=>''Int'',''quantization''=>''Int'',''use_behavioral_HDL''=>''Int'',''use_rpm''=>''String'',''block_type''=>''String''}';
      |   ptable_ = xlblockprep(get_param(tmp_gcb, 'MaskWSVariables'));
      |   try
      |     xlBlockMoveCallback(tmp_gcbh);
      |   catch 
      |      clear global xl_updateicon_recursion_guard;
      |   end;
      | catch
      |   global dbgsysgen;
      |   if(~isempty(dbgsysgen) && dbgsysgen)
      |     e = regexprep(lasterr, '\n', '\nError: ');
      |     disp(['Error: While running MaskInit code on block ' tmp_gcb ': ' e]);
      |     error(e);
      |   end
      | end
      settings: CopyFcn=xlBlockMoveCallback(gcbh);  DeleteFcn=xlDestroyGui(gcbh);  ModelCloseFcn=xlDestroyGui(gcbh);  PreSaveFcn=xlBlockPreSaveCallback(gcbh);  PostSaveFcn=xlBlockPostSaveCallback(gcbh);  DestroyFcn=xlDestroyGui(gcbh);  OpenFcn=xlOpenGui(gcbh, 'cmult_gui.xml', @cmultenablement, @cmultaction)  CloseFcn=xlDestroyGui(gcbh);  MoveFcn=xlBlockMoveCallback(gcbh);
      mask Help: eval('');xlDoc('-book','sysgen','-topic','CMult');
      mask StyleString: edit,edit,popup(Fixed-point|Floating-point),edit,edit,edit,popup(Single|Double|Custom),edit,edit,edit,checkbox,edit,edit,popup(Full|User Defined),edit,popup(Signed  (2's comp)|Unsigned),edit,edit,edit,popup(Truncate|Round  (unbiased: +/- Inf)),edit,popup(Wrap|Saturate|Flag as error),edit,checkbox,edit,checkbox,edit,popup(Distributed RAM|Block RAM),edit,checkbox,edit,checkbox,edit,edit,edit,edit,edit,edit,edit,edit,edit,edit,edit,edit
      mask Display:
      | fprintf('','COMMENT: begin icon graphics');
      | patch([0 65 0 0 ],[0 30 60 0 ],[0.77 0.82 0.91 ]);
      | plot([0 65 0 0 ],[0 30 60 0 ]);
      | patch([5.07 12.006 16.806 21.606 26.406 16.806 9.87 5.07 ],[35.328 35.328 40.128 35.328 40.128 40.128 40.128 35.328 ],[1 1 1 ]);
      | patch([9.87 16.806 12.006 5.07 9.87 ],[30.528 30.528 35.328 35.328 30.528 ],[0.931 0.946 0.973 ]);
      | patch([5.07 12.006 16.806 9.87 5.07 ],[25.728 25.728 30.528 30.528 25.728 ],[1 1 1 ]);
      | patch([9.87 26.406 21.606 16.806 12.006 5.07 9.87 ],[20.928 20.928 25.728 20.928 25.728 25.728 20.928 ],[0.931 0.946 0.973 ]);
      | fprintf('','COMMENT: end icon graphics');
      | fprintf('','COMMENT: begin icon text');
      | 
      | 
      | color('black');disp('\bf{x 1}','texmode','on');
      | fprintf('','COMMENT: end icon text');
  "CORDIC 4.0 " : S-Function  LoadFcn=xlBlockLoadCallback(gcbh);  FunctionName=sysgen  Parameters=ptable_  EnableBusSupport=off  mask(Xilinx CORDIC 4.0 Block){functional_selection=Square_Root, architectural_configuration=Parallel, pipelining_mode=Maximum, data_format=UnsignedFraction, phase_format=Radians, output_width=16, round_mode=Truncate, iterations=0, precision=0, coarse_rotation=on, compensation_scaling=No_Scale_Compensation, ce=off, sclr=off, nd=off, rdy=off, x_out=on, y_out=on, phase_output=off, xl_use_area=off, xl_area=[0,0,0,0,0,0,0], register_inputs=true, register_outputs=true, ipcore_usecache=true, ipcore_useipmodelcache=true, ipcore_verbose=false, wrapper_available=true, ip_name=CORDIC, ip_version=4.0, dsptool_ready=true, port_translation_map={ 'ce' => 'en', 'sclr' => 'rst' }, structural_sim=false, has_advanced_control=0, sggui_pos=-1,-1,-1,-1, block_type=cordic_v4_0, block_version=, sg_icon_stat=95,142,1,1,white,blue,0,4592ed88,right,,[ ],[ ], sg_mask_display=|, sg_list_contents=, sg_blockgui_xml=}
      mask sg_mask_display=|
      | fprintf('','COMMENT: begin icon graphics');
      | patch([0 95 95 0 0 ],[0 0 142 142 0 ],[0.77 0.82 0.91 ]);
      | plot([0 95 95 0 0 ],[0 0 142 142 0 ]);
      | patch([18.075 36.86 49.86 62.86 75.86 49.86 31.075 18.075 ],[85.43 85.43 98.43 85.43 98.43 98.43 98.43 85.43 ],[1 1 1 ]);
      | patch([31.075 49.86 36.86 18.075 31.075 ],[72.43 72.43 85.43 85.43 72.43 ],[0.931 0.946 0.973 ]);
      | patch([18.075 36.86 49.86 31.075 18.075 ],[59.43 59.43 72.43 72.43 59.43 ],[1 1 1 ]);
      | patch([31.075 75.86 62.86 49.86 36.86 18.075 31.075 ],[46.43 46.43 59.43 46.43 59.43 59.43 46.43 ],[0.931 0.946 0.973 ]);
      | fprintf('','COMMENT: end icon graphics');
      | fprintf('','COMMENT: begin icon text');
      | color('black');port_label('input',1,'x_in');
      | color('black');port_label('output',1,'x_out');
      | fprintf('','COMMENT: end icon text');
      mask prompts: functional_selection ""; architectural_configuration ""; pipelining_mode ""; data_format ""; phase_format ""; output_width "Output width"; round_mode ""; coarse_rotation "Coarse rotation"; compensation_scaling "Compensation scaling"; ce "en"; sclr "rst"; x_out "X out"; y_out "Y out"; phase_output "Phase output"; xl_use_area "Define FPGA area for resource estimation"; xl_area "FPGA area [slices, FFs, BRAMs, LUTs, IOBs, emb. mults, TBUFs]"; register_inputs ""; register_outputs ""; ipcore_usecache ""; ipcore_useipmodelcache ""; ipcore_verbose ""; wrapper_available ""; ip_name ""; ip_version ""; dsptool_ready ""; port_translation_map ""; structural_sim ""; has_advanced_control ""; sggui_pos ""; block_type ""; block_version ""; sg_icon_stat ""; sg_mask_display ""; sg_list_contents ""; sg_blockgui_xml ""
      mask help: Xilinx CORDIC 4.0
      mask init:
      | try
      |   tmp_gcb = gcb;
      |   tmp_gcbh = gcbh;
      |   if (strcmp('SysGenIndex',get_param(bdroot(tmp_gcbh),'tag')) && ~isempty(regexp(bdroot(tmp_gcb), '^xbs', 'once')))
      |     return;
      |   end;
      |   xlMungeMaskParams;
      |   block_config = 'sysgen:coregenimport_config';
      | 
      |   block_type='cordic_v4_0';
      | 
      |   serialized_declarations = '{''architectural_configuration''=>''String'',''ce''=>''Bool'',''coarse_rotation''=>''Bool'',''compensation_scaling''=>''String'',''data_format''=>''String'',''dsptool_ready''=>''Bool'',''functional_selection''=>''String'',''ip_name''=>''String'',''ip_version''=>''String'',''ipcore_usecache''=>''Bool'',''ipcore_useipmodelcache''=>''Bool'',''ipcore_verbose''=>''Bool'',''iterations''=>''Int'',''nd''=>''Bool'',''output_width''=>''Int'',''phase_format''=>''String'',''phase_output''=>''Bool'',''pipelining_mode''=>''String'',''port_translation_map''=>''String'',''precision''=>''Int'',''rdy''=>''Bool'',''register_inputs''=>''Bool'',''register_outputs''=>''Bool'',''round_mode''=>''String'',''sclr''=>''Bool'',''structural_sim''=>''Bool'',''wrapper_available''=>''Bool'',''x_out''=>''Bool'',''xl_use_area''=>''Bool'',''y_out''=>''Bool'',''block_type''=>''String''}';
      |   ptable_ = xlblockprep(get_param(tmp_gcb, 'MaskWSVariables'));
      |   try
      |     xlBlockMoveCallback(tmp_gcbh);
      |   catch 
      |      clear global xl_updateicon_recursion_guard;
      |   end;
      | catch
      |   global dbgsysgen;
      |   if(~isempty(dbgsysgen) && dbgsysgen)
      |     e = regexprep(lasterr, '\n', '\nError: ');
      |     disp(['Error: While running MaskInit code on block ' tmp_gcb ': ' e]);
      |     error(e);
      |   end
      | end
      settings: CopyFcn=xlBlockMoveCallback(gcbh);  DeleteFcn=xlDestroyGui(gcbh);  ModelCloseFcn=xlDestroyGui(gcbh);  PreSaveFcn=xlBlockPreSaveCallback(gcbh);  PostSaveFcn=xlBlockPostSaveCallback(gcbh);  DestroyFcn=xlDestroyGui(gcbh);  OpenFcn=xlOpenGui(gcbh, 'cordic_v4_0_gui.xml', @xlipmagiccallback_pass_evaluate_params, @xlipmagicaction)  CloseFcn=xlDestroyGui(gcbh);  MoveFcn=xlBlockMoveCallback(gcbh);
      mask Help: eval('');xlDoc('-book','sysgen','-topic','CORDIC_4_0');
      mask StyleString: popup(Rotate|Translate|Sin_and_Cos|Sinh_and_Cosh|Arc_Tan|Arc_Tanh|Square_Root),popup(Word_Serial|Parallel),popup(No_Pipelining|Optimal|Maximum),popup(SignedFraction|UnsignedFraction|UnsignedInteger),popup(Radians|Scaled_Radians),edit,popup(Truncate|Round_Pos_Inf|Round_Pos_Neg_Inf|Nearest_Even),edit,edit,checkbox,popup(No_Scale_Compensation|LUT_based|BRAM|Embedded_Multiplier),checkbox,checkbox,checkbox,checkbox,checkbox,checkbox,checkbox,checkbox,edit,edit,edit,edit,edit,edit,edit,edit,edit,edit,edit,edit,edit,edit,edit,edit,edit,edit,edit,edit
      mask Display:
      | fprintf('','COMMENT: begin icon graphics');
      | patch([0 95 95 0 0 ],[0 0 142 142 0 ],[0.77 0.82 0.91 ]);
      | plot([0 95 95 0 0 ],[0 0 142 142 0 ]);
      | patch([18.075 36.86 49.86 62.86 75.86 49.86 31.075 18.075 ],[85.43 85.43 98.43 85.43 98.43 98.43 98.43 85.43 ],[1 1 1 ]);
      | patch([31.075 49.86 36.86 18.075 31.075 ],[72.43 72.43 85.43 85.43 72.43 ],[0.931 0.946 0.973 ]);
      | patch([18.075 36.86 49.86 31.075 18.075 ],[59.43 59.43 72.43 72.43 59.43 ],[1 1 1 ]);
      | patch([31.075 75.86 62.86 49.86 36.86 18.075 31.075 ],[46.43 46.43 59.43 46.43 59.43 59.43 46.43 ],[0.931 0.946 0.973 ]);
      | fprintf('','COMMENT: end icon graphics');
      | fprintf('','COMMENT: begin icon text');
      | color('black');port_label('input',1,'x_in');
      | color('black');port_label('output',1,'x_out');
      | fprintf('','COMMENT: end icon text');
  "CORDIC 5.0 " : S-Function  LoadFcn=xlBlockLoadCallback(gcbh);  FunctionName=sysgen  Parameters=ptable_  EnableBusSupport=off  mask(Xilinx CORDIC 5.0 Block){infoedit=CORDIC 5.0, functional_selection=Rotate, architectural_configuration=Parallel, pipelining_mode=Maximum, data_format=SignedFraction, phase_format=Radians, input_width=16, output_width=16, round_mode=Truncate, iterations=0, precision=0, compensation_scaling=No_Scale_Compensation, coarse_rotation=on, aclken=off, aresetn=off, out_tready=off, cartesian_has_tuser=off, cartesian_has_tlast=off, cartesian_tuser_width=1, phase_has_tuser=off, phase_has_tlast=off, phase_tuser_width=1, out_tlast_behv=Null, flow_control=NonBlocking, optimize_goal=Resources, trim_axipin_name=on, xl_use_area=off, xl_area=[0,0,0,0,0,0,0], ip_name=CORDIC, ip_version=5.0, dsptool_ready=true, ipcore_usecache=true, ipcore_useipmodelcache=true, wrapper_available=true, port_translation_map={ 'aclken' => 'en', 'aresetn' => 'rst' }, has_advanced_control=0, sggui_pos=-1,-1,-1,-1, block_type=cordic_v5_0, block_version=, sg_icon_stat=95,142,5,3,white,blue,0,66baf398,right,,[2 2 2 3 3 ],[4 4 4 ], sg_mask_display=|, sg_list_contents=, sg_blockgui_xml=}
      mask sg_mask_display=|
      | fprintf('','COMMENT: begin icon graphics');
      | patch([0 0 2 2 ],[142 60 60 142 ],[6.025000e-001 6.400000e-001 7.075000e-001 ]);
      | patch([0 0 2 2 ],[52 0 0 52 ],[4.350000e-001 4.600000e-001 5.050000e-001 ]);
      | patch([93 93 95 95 ],[132 10 10 132 ],[2.675000e-001 2.800000e-001 3.025000e-001 ]);
      | patch([2 92 92 2 2 ],[0 0 142 142 0 ],[7.700000e-001 8.200000e-001 9.100000e-001 ]);
      | plot([2 92 92 2 2 ],[0 0 142 142 0 ]);
      |
      |
      | patch([18.075 36.86 49.86 62.86 75.86 49.86 31.075 18.075 ],[85.43 85.43 98.43 85.43 98.43 98.43 98.43 85.43 ],[1 1 1 ]);
      | patch([31.075 49.86 36.86 18.075 31.075 ],[72.43 72.43 85.43 85.43 72.43 ],[0.931 0.946 0.973 ]);
      | patch([18.075 36.86 49.86 31.075 18.075 ],[59.43 59.43 72.43 72.43 59.43 ],[1 1 1 ]);
      | patch([31.075 75.86 62.86 49.86 36.86 18.075 31.075 ],[46.43 46.43 59.43 46.43 59.43 59.43 46.43 ],[0.931 0.946 0.973 ]);
      | fprintf('','COMMENT: end icon graphics');
      | fprintf('','COMMENT: begin icon text');
      | color('black');port_label('input',1,'  cartesian_tvalid  ');
      | color('black');port_label('input',2,'  cartesian_tdata_imag  ');
      | color('black');port_label('input',3,'  cartesian_tdata_real  ');
      | color('black');port_label('input',4,'  phase_tvalid  ');
      | color('black');port_label('input',5,'  phase_tdata_phase  ');
      | color('black');port_label('output',1,'  dout_tvalid  ');
      | color('black');port_label('output',2,'  dout_tdata_imag  ');
      | color('black');port_label('output',3,'  dout_tdata_real  ');
      | fprintf('','COMMENT: end icon text');
      mask prompts: infoedit ""; functional_selection "Function"; architectural_configuration "Configuration"; pipelining_mode "Pipeline"; data_format "Data format"; phase_format "Phase format"; input_width "Input width"; output_width "Output width"; round_mode "Round"; compensation_scaling "Compensation scaling"; coarse_rotation "Course rotation"; out_tready "tready"; cartesian_has_tuser "tuser"; cartesian_has_tlast "tlast"; cartesian_tuser_width "tuser width"; phase_has_tuser "tuser"; phase_has_tlast "tlast"; phase_tuser_width "tuser width"; out_tlast_behv "Tlast behaviour"; flow_control "AXI behaviour"; optimize_goal "Optimization"; trim_axipin_name "Display shortened port names"; xl_use_area "Define FPGA area for resource estimation"; xl_area "FPGA area [slices, FFs, BRAMs, LUTs, IOBs, emb. mults, TBUFs]"; ip_name ""; ip_version ""; dsptool_ready ""; ipcore_usecache ""; ipcore_useipmodelcache ""; wrapper_available ""; port_translation_map ""; has_advanced_control ""; sggui_pos ""; block_type ""; block_version ""; sg_icon_stat ""; sg_mask_display ""; sg_list_contents ""; sg_blockgui_xml ""
      mask help: CORDIC 5.0
      mask init:
      | try
      |   tmp_gcb = gcb;
      |   tmp_gcbh = gcbh;
      |   if (strcmp('SysGenIndex',get_param(bdroot(tmp_gcbh),'tag')) && ~isempty(regexp(bdroot(tmp_gcb), '^xbs', 'once')))
      |     return;
      |   end;
      |   xlMungeMaskParams;
      |   block_config = 'sysgen:coregenimport_config';
      | 
      |   block_type='cordic_v5_0';
      | 
      |   serialized_declarations = '{''aclken''=>''Bool'',''architectural_configuration''=>''String'',''aresetn''=>''Bool'',''cartesian_has_tlast''=>''Bool'',''cartesian_has_tuser''=>''Bool'',''cartesian_tuser_width''=>''Int'',''coarse_rotation''=>''Bool'',''compensation_scaling''=>''String'',''data_format''=>''String'',''dsptool_ready''=>''Bool'',''flow_control''=>''String'',''functional_selection''=>''String'',''input_width''=>''Int'',''ip_name''=>''String'',''ip_version''=>''String'',''ipcore_usecache''=>''Bool'',''ipcore_useipmodelcache''=>''Bool'',''iterations''=>''Int'',''optimize_goal''=>''String'',''out_tlast_behv''=>''String'',''out_tready''=>''Bool'',''output_width''=>''Int'',''phase_format''=>''String'',''phase_has_tlast''=>''Bool'',''phase_has_tuser''=>''Bool'',''phase_tuser_width''=>''Int'',''pipelining_mode''=>''String'',''port_translation_map''=>''String'',''precision''=>''Int'',''round_mode''=>''String'',''trim_axipin_name''=>''Int'',''wrapper_available''=>''Bool'',''xl_use_area''=>''Bool'',''block_type''=>''String''}';
      |   ptable_ = xlblockprep(get_param(tmp_gcb, 'MaskWSVariables'));
      |   try
      |     xlBlockMoveCallback(tmp_gcbh);
      |   catch 
      |      clear global xl_updateicon_recursion_guard;
      |   end;
      | catch
      |   global dbgsysgen;
      |   if(~isempty(dbgsysgen) && dbgsysgen)
      |     e = regexprep(lasterr, '\n', '\nError: ');
      |     disp(['Error: While running MaskInit code on block ' tmp_gcb ': ' e]);
      |     error(e);
      |   end
      | end
      settings: CopyFcn=xlBlockMoveCallback(gcbh);  DeleteFcn=xlDestroyGui(gcbh);  ModelCloseFcn=xlDestroyGui(gcbh);  PreSaveFcn=xlBlockPreSaveCallback(gcbh);  PostSaveFcn=xlBlockPostSaveCallback(gcbh);  DestroyFcn=xlDestroyGui(gcbh);  OpenFcn=xlOpenGui(gcbh, 'cordic_v5_0_gui.xml', @xlipmagiccallback_pass_evaluate_params, -1)  CloseFcn=xlDestroyGui(gcbh);  MoveFcn=xlBlockMoveCallback(gcbh);
      mask Help: eval('');xlDoc('-book','sysgen','-topic','CORDIC_5_0');
      mask StyleString: edit,popup(Rotate|Translate|Sin_and_Cos|Sinh_and_Cosh|Arc_Tan|Arc_Tanh|Square_Root),popup(Word_Serial|Parallel),popup(No_Pipelining|Optimal|Maximum),popup(SignedFraction|UnsignedFraction|UnsignedInteger),popup(Radians|Scaled_Radians),edit,edit,popup(Truncate|Round_Pos_Inf|Round_Pos_Neg_Inf|Nearest_Even),edit,edit,popup(No_Scale_Compensation|LUT_based|BRAM|Embedded_Multiplier),checkbox,checkbox,checkbox,checkbox,checkbox,checkbox,edit,checkbox,checkbox,edit,popup(Null|Pass_Cartesian_TLAST|Pass_Phase_TLAST|OR_all_TLASTs|AND_all_TLASTs),popup(NonBlocking|Blocking),popup(Resources|Performance),checkbox,checkbox,edit,edit,edit,edit,edit,edit,edit,edit,edit,edit,edit,edit,edit,edit,edit,edit
      mask Display:
      | fprintf('','COMMENT: begin icon graphics');
      | patch([0 0 2 2 ],[142 60 60 142 ],[6.025000e-001 6.400000e-001 7.075000e-001 ]);
      | patch([0 0 2 2 ],[52 0 0 52 ],[4.350000e-001 4.600000e-001 5.050000e-001 ]);
      | patch([93 93 95 95 ],[132 10 10 132 ],[2.675000e-001 2.800000e-001 3.025000e-001 ]);
      | patch([2 92 92 2 2 ],[0 0 142 142 0 ],[7.700000e-001 8.200000e-001 9.100000e-001 ]);
      | plot([2 92 92 2 2 ],[0 0 142 142 0 ]);
      | 
      | 
      | patch([18.075 36.86 49.86 62.86 75.86 49.86 31.075 18.075 ],[85.43 85.43 98.43 85.43 98.43 98.43 98.43 85.43 ],[1 1 1 ]);
      | patch([31.075 49.86 36.86 18.075 31.075 ],[72.43 72.43 85.43 85.43 72.43 ],[0.931 0.946 0.973 ]);
      | patch([18.075 36.86 49.86 31.075 18.075 ],[59.43 59.43 72.43 72.43 59.43 ],[1 1 1 ]);
      | patch([31.075 75.86 62.86 49.86 36.86 18.075 31.075 ],[46.43 46.43 59.43 46.43 59.43 59.43 46.43 ],[0.931 0.946 0.973 ]);
      | fprintf('','COMMENT: end icon graphics');
      | fprintf('','COMMENT: begin icon text');
      | color('black');port_label('input',1,'  cartesian_tvalid  ');
      | color('black');port_label('input',2,'  cartesian_tdata_imag  ');
      | color('black');port_label('input',3,'  cartesian_tdata_real  ');
      | color('black');port_label('input',4,'  phase_tvalid  ');
      | color('black');port_label('input',5,'  phase_tdata_phase  ');
      | color('black');port_label('output',1,'  dout_tvalid  ');
      | color('black');port_label('output',2,'  dout_tdata_imag  ');
      | color('black');port_label('output',3,'  dout_tdata_real  ');
      | fprintf('','COMMENT: end icon text');
  ChipScope : S-Function  LoadFcn=xlBlockLoadCallback(gcbh);  FunctionName=sysgen  Parameters=ptable_  EnableBusSupport=off  mask(Xilinx ChipScope Block){infoedit=Enables run-time debugging and verification of signals by inserting ChipScope Pro ICON and ILA cores.<br><br>  Restrictions: <br>Only one ChipScope core can be instantiated in a System Generator design. A design or subsystem containing a ChipScope block must have at least one output port., num_trig_ports_sgadvanced=, num_trig_ports=2, current_port=0, show_trig_port_sgadvanced=, show_trig_port=0, match_units_sgadvanced=, match_units=1, match_type_sgadvanced=, match_type=Basic, data_is_trigger_sgadvanced=, data_is_trigger=off, num_data_ports=1, data_depth_sgadvanced=, data_depth=512, SRL16s_sgadvanced=, SRL16s=on, add_bufg_sgadvanced=, add_bufg=on, match_type_t0=1, match_type_t1=1, match_type_t2=1, match_type_t3=1, match_type_t4=1, match_type_t5=1, match_type_t6=1, match_type_t7=1, match_type_t8=1, match_type_t9=1, match_type_t10=1, match_type_t11=1, match_type_t12=1, match_type_t13=1, match_type_t14=1, match_type_t15=1, match_units_t0=1, match_units_t1=1, match_units_t2=1, match_units_t3=1, match_units_t4=1, match_units_t5=1, match_units_t6=1, match_units_t7=1, match_units_t8=1, match_units_t9=1, match_units_t10=1, match_units_t11=1, match_units_t12=1, match_units_t13=1, match_units_t14=1, match_units_t15=1, dbl_ovrd=0, user_scan_chain=USER1, has_advanced_control=0, sggui_pos=-1,-1,-1,-1, block_type=chipscope, block_version=, sg_icon_stat=60,84,3,0,white,blue,0,284c7683,right,,[ ],[ ], sg_mask_display=|, sg_list_contents=, sg_blockgui_xml=}
      mask sg_mask_display=|
      | fprintf('','COMMENT: begin icon graphics');
      | patch([0 60 60 0 0 ],[0 0 84 84 0 ],[0.77 0.82 0.91 ]);
      | plot([0 60 60 0 0 ],[0 0 84 84 0 ]);
      | patch([12.2 23.76 31.76 39.76 47.76 31.76 20.2 12.2 ],[50.88 50.88 58.88 50.88 58.88 58.88 58.88 50.88 ],[1 1 1 ]);
      | patch([20.2 31.76 23.76 12.2 20.2 ],[42.88 42.88 50.88 50.88 42.88 ],[0.931 0.946 0.973 ]);
      | patch([12.2 23.76 31.76 20.2 12.2 ],[34.88 34.88 42.88 42.88 34.88 ],[1 1 1 ]);
      | patch([20.2 47.76 39.76 31.76 23.76 12.2 20.2 ],[26.88 26.88 34.88 26.88 34.88 34.88 26.88 ],[0.931 0.946 0.973 ]);
      | fprintf('','COMMENT: end icon graphics');
      | fprintf('','COMMENT: begin icon text');
      | color('black');port_label('input',1,'trig0');
      | color('black');port_label('input',2,'trig1');
      | color('black');port_label('input',3,'data0');
      | fprintf('','COMMENT: end icon text');
      mask prompts: infoedit ""; num_trig_ports_sgadvanced ""; num_trig_ports "Number of trigger ports"; current_port ""; show_trig_port_sgadvanced ""; show_trig_port "Display settings for trigger port"; match_units_sgadvanced ""; match_units "Number of match units"; match_type_sgadvanced ""; match_type "Match type"; data_is_trigger_sgadvanced ""; data_is_trigger "Use trigger ports as data"; num_data_ports "Number of data ports"; data_depth_sgadvanced ""; data_depth "Depth of capture buffer"; SRL16s_sgadvanced ""; SRL16s "Use SRL16s (when possible)"; add_bufg_sgadvanced ""; add_bufg "Add BUFG to JTAG clock"; match_type_t0 ""; match_type_t1 ""; match_type_t2 ""; match_type_t3 ""; match_type_t4 ""; match_type_t5 ""; match_type_t6 ""; match_type_t7 ""; match_type_t8 ""; match_type_t9 ""; match_type_t10 ""; match_type_t11 ""; match_type_t12 ""; match_type_t13 ""; match_type_t14 ""; match_type_t15 ""; match_units_t0 ""; match_units_t1 ""; match_units_t2 ""; match_units_t3 ""; match_units_t4 ""; match_units_t5 ""; match_units_t6 ""; match_units_t7 ""; match_units_t8 ""; match_units_t9 ""; match_units_t10 ""; match_units_t11 ""; match_units_t12 ""; match_units_t13 ""; match_units_t14 ""; match_units_t15 ""; dbl_ovrd ""; user_scan_chain ""; has_advanced_control ""; sggui_pos ""; block_type ""; block_version ""; sg_icon_stat ""; sg_mask_display ""; sg_list_contents ""; sg_blockgui_xml ""
      mask help:
      | Enables run-time debugging and verification of signals by inserting ChipScope Pro ICON and ILA cores.
      |
      |   Restrictions:
      | Only one ChipScope core can be instantiated in a System Generator design. A design or subsystem containing a ChipScope block must have at least one output port.
      mask init:
      | try
      |   tmp_gcb = gcb;
      |   tmp_gcbh = gcbh;
      |   if (strcmp('SysGenIndex',get_param(bdroot(tmp_gcbh),'tag')) && ~isempty(regexp(bdroot(tmp_gcb), '^xbs', 'once')))
      |     return;
      |   end;
      |   xlMungeMaskParams;
      |   block_config = 'sysgen_blockset:Chipscope_config';
      | 
      |   block_type='chipscope';
      | 
      |   serialized_declarations = '{''SRL16s''=>''Int'',''add_bufg''=>''Int'',''data_depth''=>''Int'',''data_is_trigger''=>''Int'',''dstr''=>''StringVector'',''match_type_t#''=>''Int'',''match_type_t0''=>''Int'',''match_type_t1''=>''Int'',''match_type_t10''=>''Int'',''match_type_t11''=>''Int'',''match_type_t12''=>''Int'',''match_type_t13''=>''Int'',''match_type_t14''=>''Int'',''match_type_t15''=>''Int'',''match_type_t2''=>''Int'',''match_type_t3''=>''Int'',''match_type_t4''=>''Int'',''match_type_t5''=>''Int'',''match_type_t6''=>''Int'',''match_type_t7''=>''Int'',''match_type_t8''=>''Int'',''match_type_t9''=>''Int'',''match_units_t#''=>''Int'',''match_units_t0''=>''Int'',''match_units_t1''=>''Int'',''match_units_t10''=>''Int'',''match_units_t11''=>''Int'',''match_units_t12''=>''Int'',''match_units_t13''=>''Int'',''match_units_t14''=>''Int'',''match_units_t15''=>''Int'',''match_units_t2''=>''Int'',''match_units_t3''=>''Int'',''match_units_t4''=>''Int'',''match_units_t5''=>''Int'',''match_units_t6''=>''Int'',''match_units_t7''=>''Int'',''match_units_t8''=>''Int'',''match_units_t9''=>''Int'',''num_data_ports''=>''Int'',''num_trig_ports''=>''Int'',''show_trig_port''=>''Int'',''user_scan_chain''=>''String'',''block_type''=>''String''}';
      |   xlchipscope_init();
      |   ptable_ = xlblockprep(get_param(tmp_gcb, 'MaskWSVariables'));
      |   try
      |     xlBlockMoveCallback(tmp_gcbh);
      |   catch 
      |      clear global xl_updateicon_recursion_guard;
      |   end;
      | catch
      |   global dbgsysgen;
      |   if(~isempty(dbgsysgen) && dbgsysgen)
      |     e = regexprep(lasterr, '\n', '\nError: ');
      |     disp(['Error: While running MaskInit code on block ' tmp_gcb ': ' e]);
      |     error(e);
      |   end
      | end
      settings: CopyFcn=xlBlockMoveCallback(gcbh);  DeleteFcn=xlDestroyGui(gcbh);  ModelCloseFcn=xlDestroyGui(gcbh);  PreSaveFcn=xlBlockPreSaveCallback(gcbh);  PostSaveFcn=xlBlockPostSaveCallback(gcbh);  DestroyFcn=xlDestroyGui(gcbh);  OpenFcn=xlOpenGui(gcbh, 'chipscope_gui.xml', @chipscopeenablement, @chipscopeaction)  CloseFcn=xlDestroyGui(gcbh);  MoveFcn=xlBlockMoveCallback(gcbh);
      mask Help: eval('');xlDoc('-book','sysgen','-topic','ChipScope');
      mask StyleString: edit,edit,popup(1|2|3|4|5|6|7|8|9|10|11|12|13|14|15|16),edit,edit,popup(0|1|2|3|4|5|6|7|8|9|10|11|12|13|14|15),edit,popup(1|2|3|4),edit,popup(Basic|Basic with edges|Extended|Extended with edges|Range|Range with edges),edit,checkbox,edit,edit,popup(512|1024|2048|4096|8192|16384|32768|65536|131072),edit,checkbox,edit,checkbox,edit,edit,edit,edit,edit,edit,edit,edit,edit,edit,edit,edit,edit,edit,edit,edit,edit,edit,edit,edit,edit,edit,edit,edit,edit,edit,edit,edit,edit,edit,edit,edit,edit,edit,edit,edit,edit,edit,edit,edit,edit,edit
      mask Display:
      | fprintf('','COMMENT: begin icon graphics');
      | patch([0 60 60 0 0 ],[0 0 84 84 0 ],[0.77 0.82 0.91 ]);
      | plot([0 60 60 0 0 ],[0 0 84 84 0 ]);
      | patch([12.2 23.76 31.76 39.76 47.76 31.76 20.2 12.2 ],[50.88 50.88 58.88 50.88 58.88 58.88 58.88 50.88 ],[1 1 1 ]);
      | patch([20.2 31.76 23.76 12.2 20.2 ],[42.88 42.88 50.88 50.88 42.88 ],[0.931 0.946 0.973 ]);
      | patch([12.2 23.76 31.76 20.2 12.2 ],[34.88 34.88 42.88 42.88 34.88 ],[1 1 1 ]);
      | patch([20.2 47.76 39.76 31.76 23.76 12.2 20.2 ],[26.88 26.88 34.88 26.88 34.88 34.88 26.88 ],[0.931 0.946 0.973 ]);
      | fprintf('','COMMENT: end icon graphics');
      | fprintf('','COMMENT: begin icon text');
      | color('black');port_label('input',1,'trig0');
      | color('black');port_label('input',2,'trig1');
      | color('black');port_label('input',3,'data0');
      | fprintf('','COMMENT: end icon text');
  Clock Enable Probe : S-Function  LoadFcn=xlBlockLoadCallback(gcbh);  FunctionName=sysgen  Parameters=ptable_  EnableBusSupport=off  mask(Xilinx Clock Enable Probe Block){infoedit=Clock enable extractor.  Produces a Boolean output that mirrors the hardware clock enable associated with the input sample rate.<br><br>Hardware notes: in hardware this block costs nothing., inherit_constraints_sgadvanced=, inherit_constraints=on, has_advanced_control=0, sggui_pos=-1,-1,-1,-1, block_type=ceprobe, block_version=, sg_icon_stat=45,28,1,1,white,blue,0,16c0cf07,right,,[ ],[ ], sg_mask_display=|, sg_list_contents=, sg_blockgui_xml=}
      mask sg_mask_display=|
      | fprintf('','COMMENT: begin icon graphics');
      | patch([0 45 45 0 0 ],[0 0 28 28 0 ],[0.77 0.82 0.91 ]);
      | plot([0 45 45 0 0 ],[0 0 28 28 0 ]);
      | patch([13.1 18.88 22.88 26.88 30.88 22.88 17.1 13.1 ],[18.44 18.44 22.44 18.44 22.44 22.44 22.44 18.44 ],[1 1 1 ]);
      | patch([17.1 22.88 18.88 13.1 17.1 ],[14.44 14.44 18.44 18.44 14.44 ],[0.931 0.946 0.973 ]);
      | patch([13.1 18.88 22.88 17.1 13.1 ],[10.44 10.44 14.44 14.44 10.44 ],[1 1 1 ]);
      | patch([17.1 30.88 26.88 22.88 18.88 13.1 17.1 ],[6.44 6.44 10.44 6.44 10.44 10.44 6.44 ],[0.931 0.946 0.973 ]);
      | fprintf('','COMMENT: end icon graphics');
      | fprintf('','COMMENT: begin icon text');
      |
      |
      | color('black');disp('CEProbe');
      | fprintf('','COMMENT: end icon text');
      mask prompts: infoedit ""; inherit_constraints_sgadvanced ""; inherit_constraints "Use clock enable signal without Multi-Cycle path constraints"; has_advanced_control ""; sggui_pos ""; block_type ""; block_version ""; sg_icon_stat ""; sg_mask_display ""; sg_list_contents ""; sg_blockgui_xml ""
      mask help:
      | Clock enable extractor.  Produces a Boolean output that mirrors the hardware clock enable associated with the input sample rate.
      |
      | Hardware notes: in hardware this block costs nothing.
      mask init:
      | try
      |   tmp_gcb = gcb;
      |   tmp_gcbh = gcbh;
      |   if (strcmp('SysGenIndex',get_param(bdroot(tmp_gcbh),'tag')) && ~isempty(regexp(bdroot(tmp_gcb), '^xbs', 'once')))
      |     return;
      |   end;
      |   xlMungeMaskParams;
      |   block_config = 'sysgen_blockset:CEProbe_config';
      | 
      |   block_type='ceprobe';
      | 
      |   serialized_declarations = '{''block_fullname''=>''String'',''enable_debug''=>''Int'',''enable_stdout''=>''Int'',''inherit_constraints''=>''Int'',''period''=>''Double'',''block_type''=>''String''}';
      |   xlceprobe_init();
      |   ptable_ = xlblockprep(get_param(tmp_gcb, 'MaskWSVariables'));
      |   try
      |     xlBlockMoveCallback(tmp_gcbh);
      |   catch 
      |      clear global xl_updateicon_recursion_guard;
      |   end;
      | catch
      |   global dbgsysgen;
      |   if(~isempty(dbgsysgen) && dbgsysgen)
      |     e = regexprep(lasterr, '\n', '\nError: ');
      |     disp(['Error: While running MaskInit code on block ' tmp_gcb ': ' e]);
      |     error(e);
      |   end
      | end
      settings: CopyFcn=xlBlockMoveCallback(gcbh);  DeleteFcn=xlDestroyGui(gcbh);  ModelCloseFcn=xlDestroyGui(gcbh);  PreSaveFcn=xlBlockPreSaveCallback(gcbh);  PostSaveFcn=xlBlockPostSaveCallback(gcbh);  DestroyFcn=xlDestroyGui(gcbh);  OpenFcn=xlOpenGui(gcbh, 'ceprobe_gui.xml', -1, -1)  CloseFcn=xlDestroyGui(gcbh);  MoveFcn=xlBlockMoveCallback(gcbh);
      mask Help: eval('');xlDoc('-book','sysgen','-topic','Clock_Enable_Probe');
      mask Display:
      | fprintf('','COMMENT: begin icon graphics');
      | patch([0 45 45 0 0 ],[0 0 28 28 0 ],[0.77 0.82 0.91 ]);
      | plot([0 45 45 0 0 ],[0 0 28 28 0 ]);
      | patch([13.1 18.88 22.88 26.88 30.88 22.88 17.1 13.1 ],[18.44 18.44 22.44 18.44 22.44 22.44 22.44 18.44 ],[1 1 1 ]);
      | patch([17.1 22.88 18.88 13.1 17.1 ],[14.44 14.44 18.44 18.44 14.44 ],[0.931 0.946 0.973 ]);
      | patch([13.1 18.88 22.88 17.1 13.1 ],[10.44 10.44 14.44 14.44 10.44 ],[1 1 1 ]);
      | patch([17.1 30.88 26.88 22.88 18.88 13.1 17.1 ],[6.44 6.44 10.44 6.44 10.44 10.44 6.44 ],[0.931 0.946 0.973 ]);
      | fprintf('','COMMENT: end icon graphics');
      | fprintf('','COMMENT: begin icon text');
      | 
      | 
      | color('black');disp('CEProbe');
      | fprintf('','COMMENT: end icon text');
  Clock Probe : Subsystem  LoadFcn=xlBlockLoadCallback(gcbh);  mask(Xilinx Clock Probe Block){infoedit=Clock probe.  Produces an output of type double that mirrors the hardware system clock.<br><br>Hardware notes:  This block is ignored when hardware is generated., has_advanced_control=0, sggui_pos=-1,-1,-1,-1, block_type=clkprobe, block_version=, sg_icon_stat=25,28,-1,-1,white,yellow,4,07734,right,,[ ],[ ], sg_mask_display=|, sg_list_contents=, sg_blockgui_xml=}
      mask sg_mask_display=|
      | fprintf('','COMMENT: begin icon graphics');
      | patch([25 24.7598 24.0485 22.8934 21.3388 19.4446 17.2835 14.9386 12.5 10.0614 7.71646 5.55537 3.66117 2.10663 0.951506 0.240184 0 0.240184 0.951506 2.10663 3.66117 5.55537 7.71646 10.0614 12.5 14.9386 17.2835 19.4446 21.3388 22.8934 24.0485 24.7598 25 25 ],[14 16.7313 19.3576 21.778 23.8995 25.6406 26.9343 27.731 28 27.731 26.9343 25.6406 23.8995 21.778 19.3576 16.7313 14 11.2687 8.64243 6.22202 4.10051 2.35943 1.06569 0.269006 0 0.269006 1.06569 2.35943 4.10051 6.22202 8.64243 11.2687 14 14 ],[0.95 0.93 0.65 ]);
      | plot([25 24.7598 24.0485 22.8934 21.3388 19.4446 17.2835 14.9386 12.5 10.0614 7.71646 5.55537 3.66117 2.10663 0.951506 0.240184 0 0.240184 0.951506 2.10663 3.66117 5.55537 7.71646 10.0614 12.5 14.9386 17.2835 19.4446 21.3388 22.8934 24.0485 24.7598 25 25 ],[14 16.7313 19.3576 21.778 23.8995 25.6406 26.9343 27.731 28 27.731 26.9343 25.6406 23.8995 21.778 19.3576 16.7313 14 11.2687 8.64243 6.22202 4.10051 2.35943 1.06569 0.269006 0 0.269006 1.06569 2.35943 4.10051 6.22202 8.64243 11.2687 14 14 ]);
      | patch([5.325 9.66 12.66 15.66 18.66 12.66 8.325 5.325 ],[17.33 17.33 20.33 17.33 20.33 20.33 20.33 17.33 ],[1 1 1 ]);
      | patch([8.325 12.66 9.66 5.325 8.325 ],[14.33 14.33 17.33 17.33 14.33 ],[0.985 0.979 0.895 ]);
      | patch([5.325 9.66 12.66 8.325 5.325 ],[11.33 11.33 14.33 14.33 11.33 ],[1 1 1 ]);
      | patch([8.325 18.66 15.66 12.66 9.66 5.325 8.325 ],[8.33 8.33 11.33 8.33 11.33 11.33 8.33 ],[0.985 0.979 0.895 ]);
      | fprintf('','COMMENT: end icon graphics');
      | fprintf('','COMMENT: begin icon text');
      | fprintf('','COMMENT: end icon text');
      mask prompts: infoedit ""; has_advanced_control ""; sggui_pos ""; block_type ""; block_version ""; sg_icon_stat ""; sg_mask_display ""; sg_list_contents ""; sg_blockgui_xml ""
      mask help:
      | Clock probe.  Produces an output of type double that mirrors the hardware system clock.
      |
      | Hardware notes:  This block is ignored when hardware is generated.
      mask init:
      | try
      |   tmp_gcb = gcb;
      |   tmp_gcbh = gcbh;
      |   if (strcmp('SysGenIndex',get_param(bdroot(tmp_gcbh),'tag')) && ~isempty(regexp(bdroot(tmp_gcb), '^xbs', 'once')))
      |     return;
      |   end;
      |   xlMungeMaskParams;
      | 
      |   block_type='clkprobe';
      | 
      |   serialized_declarations = '{''period''=>''Double'',''block_type''=>''String''}';
      |   xlclkprobe_init();
      |   ptable_ = xlblockprep(get_param(tmp_gcb, 'MaskWSVariables'));
      |   try
      |     xlBlockMoveCallback(tmp_gcbh);
      |   catch 
      |      clear global xl_updateicon_recursion_guard;
      |   end;
      | catch
      |   global dbgsysgen;
      |   if(~isempty(dbgsysgen) && dbgsysgen)
      |     e = regexprep(lasterr, '\n', '\nError: ');
      |     disp(['Error: While running MaskInit code on block ' tmp_gcb ': ' e]);
      |     error(e);
      |   end
      | end
      settings: CopyFcn=xlBlockMoveCallback(gcbh);  DeleteFcn=xlDestroyGui(gcbh);  ModelCloseFcn=xlDestroyGui(gcbh);  PreSaveFcn=xlBlockPreSaveCallback(gcbh);  PostSaveFcn=xlBlockPostSaveCallback(gcbh);  DestroyFcn=xlDestroyGui(gcbh);  OpenFcn=xlOpenGui(gcbh, 'clkprobe_gui.xml', -1, -1)  CloseFcn=xlDestroyGui(gcbh);  MoveFcn=xlBlockMoveCallback(gcbh);
      mask Help: eval('');xlDoc('-book','sysgen','-topic','Clock_Probe');
      mask Display:
      | fprintf('','COMMENT: begin icon graphics');
      | patch([25 24.7598 24.0485 22.8934 21.3388 19.4446 17.2835 14.9386 12.5 10.0614 7.71646 5.55537 3.66117 2.10663 0.951506 0.240184 0 0.240184 0.951506 2.10663 3.66117 5.55537 7.71646 10.0614 12.5 14.9386 17.2835 19.4446 21.3388 22.8934 24.0485 24.7598 25 25 ],[14 16.7313 19.3576 21.778 23.8995 25.6406 26.9343 27.731 28 27.731 26.9343 25.6406 23.8995 21.778 19.3576 16.7313 14 11.2687 8.64243 6.22202 4.10051 2.35943 1.06569 0.269006 0 0.269006 1.06569 2.35943 4.10051 6.22202 8.64243 11.2687 14 14 ],[0.95 0.93 0.65 ]);
      | plot([25 24.7598 24.0485 22.8934 21.3388 19.4446 17.2835 14.9386 12.5 10.0614 7.71646 5.55537 3.66117 2.10663 0.951506 0.240184 0 0.240184 0.951506 2.10663 3.66117 5.55537 7.71646 10.0614 12.5 14.9386 17.2835 19.4446 21.3388 22.8934 24.0485 24.7598 25 25 ],[14 16.7313 19.3576 21.778 23.8995 25.6406 26.9343 27.731 28 27.731 26.9343 25.6406 23.8995 21.778 19.3576 16.7313 14 11.2687 8.64243 6.22202 4.10051 2.35943 1.06569 0.269006 0 0.269006 1.06569 2.35943 4.10051 6.22202 8.64243 11.2687 14 14 ]);
      | patch([5.325 9.66 12.66 15.66 18.66 12.66 8.325 5.325 ],[17.33 17.33 20.33 17.33 20.33 20.33 20.33 17.33 ],[1 1 1 ]);
      | patch([8.325 12.66 9.66 5.325 8.325 ],[14.33 14.33 17.33 17.33 14.33 ],[0.985 0.979 0.895 ]);
      | patch([5.325 9.66 12.66 8.325 5.325 ],[11.33 11.33 14.33 14.33 11.33 ],[1 1 1 ]);
      | patch([8.325 18.66 15.66 12.66 9.66 5.325 8.325 ],[8.33 8.33 11.33 8.33 11.33 11.33 8.33 ],[0.985 0.979 0.895 ]);
      | fprintf('','COMMENT: end icon graphics');
      | fprintf('','COMMENT: begin icon text');
      | fprintf('','COMMENT: end icon text');
  "Complex Multiplier 3.0 " : S-Function  LoadFcn=xlBlockLoadCallback(gcbh);  FunctionName=sysgen  Parameters=ptable_  EnableBusSupport=off  mask(Xilinx Complex Multiplier 3.0 Block){multtype=Use_Mults, optimizegoal=Resources, outputwidthhigh=32, outputwidthlow=0, roundmode=Truncate, clockenable=off, syncclear=off, xl_use_area=off, xl_area=[0,0,0,0,0,0,0], ip_name=Complex Multiplier, ip_version=3.0, dsptool_ready=true, ipcore_usecache=true, ipcore_useipmodelcache=true, ipcore_verbose=false, wrapper_available=true, port_translation_map={ 'ce' => 'en', 'sclr' => 'rst' }, structural_sim=false, has_advanced_control=0, sggui_pos=-1,-1,-1,-1, block_type=cmpy_v3_0, block_version=, sg_icon_stat=95,143,4,2,white,blue,0,326efc33,right,,[ ],[ ], sg_mask_display=|, sg_list_contents=, sg_blockgui_xml=}
      mask sg_mask_display=|
      | fprintf('','COMMENT: begin icon graphics');
      | patch([0 95 95 0 0 ],[0 0 143 143 0 ],[0.77 0.82 0.91 ]);
      | plot([0 95 95 0 0 ],[0 0 143 143 0 ]);
      | patch([18.075 36.86 49.86 62.86 75.86 49.86 31.075 18.075 ],[85.43 85.43 98.43 85.43 98.43 98.43 98.43 85.43 ],[1 1 1 ]);
      | patch([31.075 49.86 36.86 18.075 31.075 ],[72.43 72.43 85.43 85.43 72.43 ],[0.931 0.946 0.973 ]);
      | patch([18.075 36.86 49.86 31.075 18.075 ],[59.43 59.43 72.43 72.43 59.43 ],[1 1 1 ]);
      | patch([31.075 75.86 62.86 49.86 36.86 18.075 31.075 ],[46.43 46.43 59.43 46.43 59.43 59.43 46.43 ],[0.931 0.946 0.973 ]);
      | fprintf('','COMMENT: end icon graphics');
      | fprintf('','COMMENT: begin icon text');
      | color('black');port_label('input',1,'ar');
      | color('black');port_label('input',2,'ai');
      | color('black');port_label('input',3,'br');
      | color('black');port_label('input',4,'bi');
      | color('black');port_label('output',1,'pr');
      | color('black');port_label('output',2,'pi');
      | fprintf('','COMMENT: end icon text');
      mask prompts: multtype ""; optimizegoal ""; outputwidthhigh "Output MSB"; outputwidthlow "Output LSB"; roundmode ""; clockenable "en"; syncclear "rst"; xl_use_area "Define FPGA area for resource estimation"; xl_area "FPGA area [slices, FFs, BRAMs, LUTs, IOBs, emb. mults, TBUFs]"; ip_name ""; ip_version ""; dsptool_ready ""; ipcore_usecache ""; ipcore_useipmodelcache ""; ipcore_verbose ""; wrapper_available ""; port_translation_map ""; structural_sim ""; has_advanced_control ""; sggui_pos ""; block_type ""; block_version ""; sg_icon_stat ""; sg_mask_display ""; sg_list_contents ""; sg_blockgui_xml ""
      mask help: Xilinx Complex Multiplier 3.0
      mask init:
      | try
      |   tmp_gcb = gcb;
      |   tmp_gcbh = gcbh;
      |   if (strcmp('SysGenIndex',get_param(bdroot(tmp_gcbh),'tag')) && ~isempty(regexp(bdroot(tmp_gcb), '^xbs', 'once')))
      |     return;
      |   end;
      |   xlMungeMaskParams;
      |   block_config = 'sysgen:coregenimport_config';
      | 
      |   block_type='cmpy_v3_0';
      | 
      |   serialized_declarations = '{''clockenable''=>''Bool'',''dsptool_ready''=>''Bool'',''ip_name''=>''String'',''ip_version''=>''String'',''ipcore_usecache''=>''Bool'',''ipcore_useipmodelcache''=>''Bool'',''ipcore_verbose''=>''Bool'',''multtype''=>''String'',''optimizegoal''=>''String'',''outputwidthhigh''=>''Int'',''outputwidthlow''=>''Int'',''port_translation_map''=>''String'',''roundmode''=>''String'',''structural_sim''=>''Bool'',''syncclear''=>''Bool'',''wrapper_available''=>''Bool'',''xl_use_area''=>''Bool'',''block_type''=>''String''}';
      |   ptable_ = xlblockprep(get_param(tmp_gcb, 'MaskWSVariables'));
      |   try
      |     xlBlockMoveCallback(tmp_gcbh);
      |   catch 
      |      clear global xl_updateicon_recursion_guard;
      |   end;
      | catch
      |   global dbgsysgen;
      |   if(~isempty(dbgsysgen) && dbgsysgen)
      |     e = regexprep(lasterr, '\n', '\nError: ');
      |     disp(['Error: While running MaskInit code on block ' tmp_gcb ': ' e]);
      |     error(e);
      |   end
      | end
      settings: CopyFcn=xlBlockMoveCallback(gcbh);  DeleteFcn=xlDestroyGui(gcbh);  ModelCloseFcn=xlDestroyGui(gcbh);  PreSaveFcn=xlBlockPreSaveCallback(gcbh);  PostSaveFcn=xlBlockPostSaveCallback(gcbh);  DestroyFcn=xlDestroyGui(gcbh);  OpenFcn=xlOpenGui(gcbh, 'cmpy_v3_0_gui.xml', @xlipmagiccallback_pass_evaluate_params, @xlipmagicaction)  CloseFcn=xlDestroyGui(gcbh);  MoveFcn=xlBlockMoveCallback(gcbh);
      mask Help: eval('');xlDoc('-book','sysgen','-topic','Complex_Multiplier_3_0');
      mask StyleString: popup(Use_LUTs|Use_Mults),popup(Resources|Performance),edit,edit,popup(Truncate|Random_Rounding),checkbox,checkbox,checkbox,edit,edit,edit,edit,edit,edit,edit,edit,edit,edit,edit,edit,edit,edit,edit,edit,edit,edit
      mask Display:
      | fprintf('','COMMENT: begin icon graphics');
      | patch([0 95 95 0 0 ],[0 0 143 143 0 ],[0.77 0.82 0.91 ]);
      | plot([0 95 95 0 0 ],[0 0 143 143 0 ]);
      | patch([18.075 36.86 49.86 62.86 75.86 49.86 31.075 18.075 ],[85.43 85.43 98.43 85.43 98.43 98.43 98.43 85.43 ],[1 1 1 ]);
      | patch([31.075 49.86 36.86 18.075 31.075 ],[72.43 72.43 85.43 85.43 72.43 ],[0.931 0.946 0.973 ]);
      | patch([18.075 36.86 49.86 31.075 18.075 ],[59.43 59.43 72.43 72.43 59.43 ],[1 1 1 ]);
      | patch([31.075 75.86 62.86 49.86 36.86 18.075 31.075 ],[46.43 46.43 59.43 46.43 59.43 59.43 46.43 ],[0.931 0.946 0.973 ]);
      | fprintf('','COMMENT: end icon graphics');
      | fprintf('','COMMENT: begin icon text');
      | color('black');port_label('input',1,'ar');
      | color('black');port_label('input',2,'ai');
      | color('black');port_label('input',3,'br');
      | color('black');port_label('input',4,'bi');
      | color('black');port_label('output',1,'pr');
      | color('black');port_label('output',2,'pi');
      | fprintf('','COMMENT: end icon text');
  "Complex Multiplier 3.1 " : S-Function  LoadFcn=xlBlockLoadCallback(gcbh);  FunctionName=sysgen  Parameters=ptable_  EnableBusSupport=off  mask(Xilinx Complex Multiplier 3.1 Block){multtype=Use_Mults, optimizegoal=Resources, outputwidthhigh=32, outputwidthlow=0, latency=-1, roundmode=Truncate, clockenable=off, syncclear=off, xl_use_area=off, xl_area=[0,0,0,0,0,0,0], ip_name=Complex Multiplier, ip_version=3.1, dsptool_ready=true, ipcore_usecache=true, ipcore_useipmodelcache=true, ipcore_verbose=false, ipcore_latency_parameter='latency', wrapper_available=true, port_translation_map={ 'ce' => 'en', 'sclr' => 'rst' }, structural_sim=false, has_advanced_control=0, sggui_pos=-1,-1,-1,-1, block_type=cmpy_v3_1, block_version=, sg_icon_stat=95,143,4,2,white,blue,0,326efc33,right,,[ ],[ ], sg_mask_display=|, sg_list_contents=, sg_blockgui_xml=}
      mask sg_mask_display=|
      | fprintf('','COMMENT: begin icon graphics');
      | patch([0 95 95 0 0 ],[0 0 143 143 0 ],[0.77 0.82 0.91 ]);
      | plot([0 95 95 0 0 ],[0 0 143 143 0 ]);
      | patch([18.075 36.86 49.86 62.86 75.86 49.86 31.075 18.075 ],[85.43 85.43 98.43 85.43 98.43 98.43 98.43 85.43 ],[1 1 1 ]);
      | patch([31.075 49.86 36.86 18.075 31.075 ],[72.43 72.43 85.43 85.43 72.43 ],[0.931 0.946 0.973 ]);
      | patch([18.075 36.86 49.86 31.075 18.075 ],[59.43 59.43 72.43 72.43 59.43 ],[1 1 1 ]);
      | patch([31.075 75.86 62.86 49.86 36.86 18.075 31.075 ],[46.43 46.43 59.43 46.43 59.43 59.43 46.43 ],[0.931 0.946 0.973 ]);
      | fprintf('','COMMENT: end icon graphics');
      | fprintf('','COMMENT: begin icon text');
      | color('black');port_label('input',1,'ar');
      | color('black');port_label('input',2,'ai');
      | color('black');port_label('input',3,'br');
      | color('black');port_label('input',4,'bi');
      | color('black');port_label('output',1,'pr');
      | color('black');port_label('output',2,'pi');
      | fprintf('','COMMENT: end icon text');
      mask prompts: multtype ""; optimizegoal ""; outputwidthhigh "Output MSB"; outputwidthlow "Output LSB"; latency "Select -1 to pipeline the core for maximum performance"; roundmode ""; clockenable "en"; syncclear "rst"; xl_use_area "Define FPGA area for resource estimation"; xl_area "FPGA area [slices, FFs, BRAMs, LUTs, IOBs, emb. mults, TBUFs]"; ip_name ""; ip_version ""; dsptool_ready ""; ipcore_usecache ""; ipcore_useipmodelcache ""; ipcore_verbose ""; ipcore_latency_parameter ""; wrapper_available ""; port_translation_map ""; structural_sim ""; has_advanced_control ""; sggui_pos ""; block_type ""; block_version ""; sg_icon_stat ""; sg_mask_display ""; sg_list_contents ""; sg_blockgui_xml ""
      mask help: Xilinx Complex Multiplier 3.1
      mask init:
      | try
      |   tmp_gcb = gcb;
      |   tmp_gcbh = gcbh;
      |   if (strcmp('SysGenIndex',get_param(bdroot(tmp_gcbh),'tag')) && ~isempty(regexp(bdroot(tmp_gcb), '^xbs', 'once')))
      |     return;
      |   end;
      |   xlMungeMaskParams;
      |   block_config = 'sysgen:coregenimport_config';
      | 
      |   block_type='cmpy_v3_1';
      | 
      |   serialized_declarations = '{''clockenable''=>''Bool'',''dsptool_ready''=>''Bool'',''ip_name''=>''String'',''ip_version''=>''String'',''ipcore_latency_parameter''=>''String'',''ipcore_usecache''=>''Bool'',''ipcore_useipmodelcache''=>''Bool'',''ipcore_verbose''=>''Bool'',''latency''=>''String'',''multtype''=>''String'',''optimizegoal''=>''String'',''outputwidthhigh''=>''Int'',''outputwidthlow''=>''Int'',''port_translation_map''=>''String'',''roundmode''=>''String'',''structural_sim''=>''Bool'',''syncclear''=>''Bool'',''wrapper_available''=>''Bool'',''xl_use_area''=>''Bool'',''block_type''=>''String''}';
      |   ptable_ = xlblockprep(get_param(tmp_gcb, 'MaskWSVariables'));
      |   try
      |     xlBlockMoveCallback(tmp_gcbh);
      |   catch 
      |      clear global xl_updateicon_recursion_guard;
      |   end;
      | catch
      |   global dbgsysgen;
      |   if(~isempty(dbgsysgen) && dbgsysgen)
      |     e = regexprep(lasterr, '\n', '\nError: ');
      |     disp(['Error: While running MaskInit code on block ' tmp_gcb ': ' e]);
      |     error(e);
      |   end
      | end
      settings: CopyFcn=xlBlockMoveCallback(gcbh);  DeleteFcn=xlDestroyGui(gcbh);  ModelCloseFcn=xlDestroyGui(gcbh);  PreSaveFcn=xlBlockPreSaveCallback(gcbh);  PostSaveFcn=xlBlockPostSaveCallback(gcbh);  DestroyFcn=xlDestroyGui(gcbh);  OpenFcn=xlOpenGui(gcbh, 'cmpy_v3_1_gui.xml', @xlipmagiccallback_pass_evaluate_params, @xlipmagicaction)  CloseFcn=xlDestroyGui(gcbh);  MoveFcn=xlBlockMoveCallback(gcbh);
      mask Help: eval('');xlDoc('-book','sysgen','-topic','Complex_Multiplier_3_1');
      mask StyleString: popup(Use_LUTs|Use_Mults),popup(Resources|Performance),edit,edit,popup(-1|0|1|2|3|4|5|6|7|8|9|10|11|12|13|14|15|16|17|18|19|20|21|22|23|24|25|26|27|28|29|30|31|32|33|34|35|36|37|38|39|40|41|42|43|44|45|46|47|48|49|50),popup(Truncate|Random_Rounding),checkbox,checkbox,checkbox,edit,edit,edit,edit,edit,edit,edit,edit,edit,edit,edit,edit,edit,edit,edit,edit,edit,edit,edit
      mask Display:
      | fprintf('','COMMENT: begin icon graphics');
      | patch([0 95 95 0 0 ],[0 0 143 143 0 ],[0.77 0.82 0.91 ]);
      | plot([0 95 95 0 0 ],[0 0 143 143 0 ]);
      | patch([18.075 36.86 49.86 62.86 75.86 49.86 31.075 18.075 ],[85.43 85.43 98.43 85.43 98.43 98.43 98.43 85.43 ],[1 1 1 ]);
      | patch([31.075 49.86 36.86 18.075 31.075 ],[72.43 72.43 85.43 85.43 72.43 ],[0.931 0.946 0.973 ]);
      | patch([18.075 36.86 49.86 31.075 18.075 ],[59.43 59.43 72.43 72.43 59.43 ],[1 1 1 ]);
      | patch([31.075 75.86 62.86 49.86 36.86 18.075 31.075 ],[46.43 46.43 59.43 46.43 59.43 59.43 46.43 ],[0.931 0.946 0.973 ]);
      | fprintf('','COMMENT: end icon graphics');
      | fprintf('','COMMENT: begin icon text');
      | color('black');port_label('input',1,'ar');
      | color('black');port_label('input',2,'ai');
      | color('black');port_label('input',3,'br');
      | color('black');port_label('input',4,'bi');
      | color('black');port_label('output',1,'pr');
      | color('black');port_label('output',2,'pi');
      | fprintf('','COMMENT: end icon text');
  "Complex Multiplier 4.0 " : S-Function  LoadFcn=xlBlockLoadCallback(gcbh);  FunctionName=sysgen  Parameters=ptable_  EnableBusSupport=off  mask(Xilinx Complex Multiplier 4.0  Block){hasatlast_sgadvanced=, hasatlast=off, hasatuser_sgadvanced=, hasatuser=off, atuserwidth=1, hasbtlast_sgadvanced=, hasbtlast=off, hasbtuser_sgadvanced=, hasbtuser=off, btuserwidth=1, multtype_sgadvanced=, multtype=Use_Mults, optimizegoal_sgadvanced=, optimizegoal=Resources, flowcontrol_sgadvanced=, flowcontrol=NonBlocking, outputwidth=33, roundmode_sgadvanced=, roundmode=Truncate, hasctrltlast_sgadvanced=, hasctrltlast=off, hasctrltuser_sgadvanced=, hasctrltuser=off, ctrltuserwidth=1, outtlastbehv=Null, latencyconfig=Automatic, minimumlatency=15, aclken_sgadvanced=, aclken=off, aresetn_sgadvanced=, aresetn=off, trim_axipin_name=on, aportwidth=63, bportwidth=63, ip_name=Complex Multiplier, ip_version=4.0, dsptool_ready=true, ipcore_usecache=true, ipcore_useipmodelcache=true, ipcore_verbose=false, wrapper_available=true, port_translation_map={ 'aclken' => 'en', 'aresetn' => 'rst'}, structural_sim=false, has_advanced_control=0, sggui_pos=-1,-1,-1,-1, block_type=cmpy_v4_0, block_version=, sg_icon_stat=135,165,6,3,white,blue,0,7e63527f,right,,[2 2 2 3 3 3 ],[4 4 4 ], sg_mask_display=|, sg_list_contents=, sg_blockgui_xml=}
      mask sg_mask_display=|
      | fprintf('','COMMENT: begin icon graphics');
      | patch([0 0 3 3 ],[154 86 86 154 ],[6.025000e-001 6.400000e-001 7.075000e-001 ]);
      | patch([0 0 3 3 ],[79 11 11 79 ],[4.350000e-001 4.600000e-001 5.050000e-001 ]);
      | patch([132 132 135 135 ],[154 6 6 154 ],[2.675000e-001 2.800000e-001 3.025000e-001 ]);
      | patch([3 131 131 3 3 ],[0 0 165 165 0 ],[7.700000e-001 8.200000e-001 9.100000e-001 ]);
      | plot([3 131 131 3 3 ],[0 0 165 165 0 ]);
      |
      |
      | patch([24.725 52.18 71.18 90.18 109.18 71.18 43.725 24.725 ],[103.09 103.09 122.09 103.09 122.09 122.09 122.09 103.09 ],[1 1 1 ]);
      | patch([43.725 71.18 52.18 24.725 43.725 ],[84.09 84.09 103.09 103.09 84.09 ],[0.931 0.946 0.973 ]);
      | patch([24.725 52.18 71.18 43.725 24.725 ],[65.09 65.09 84.09 84.09 65.09 ],[1 1 1 ]);
      | patch([43.725 109.18 90.18 71.18 52.18 24.725 43.725 ],[46.09 46.09 65.09 46.09 65.09 65.09 46.09 ],[0.931 0.946 0.973 ]);
      | fprintf('','COMMENT: end icon graphics');
      | fprintf('','COMMENT: begin icon text');
      | color('black');port_label('input',1,'  a_tvalid  ');
      | color('black');port_label('input',2,'  a_tdata_imag  ');
      | color('black');port_label('input',3,'  a_tdata_real  ');
      | color('black');port_label('input',4,'  b_tvalid  ');
      | color('black');port_label('input',5,'  b_tdata_imag  ');
      | color('black');port_label('input',6,'  b_tdata_real  ');
      | color('black');port_label('output',1,'  dout_tvalid  ');
      | color('black');port_label('output',2,'  dout_tdata_imag  ');
      | color('black');port_label('output',3,'  dout_tdata_real  ');
      | fprintf('','COMMENT: end icon text');
      mask prompts: hasatlast_sgadvanced ""; hasatlast "Has TLAST"; hasatuser_sgadvanced ""; hasatuser "Has TUSER"; atuserwidth "TUSER Width"; hasbtlast_sgadvanced ""; hasbtlast "Has TLAST"; hasbtuser_sgadvanced ""; hasbtuser "Has TUSER"; btuserwidth "TUSER Width"; multtype_sgadvanced ""; multtype ""; optimizegoal_sgadvanced ""; optimizegoal ""; flowcontrol_sgadvanced ""; flowcontrol ""; outputwidth "Output Width"; roundmode_sgadvanced ""; roundmode ""; hasctrltlast_sgadvanced ""; hasctrltlast "Has TLAST"; hasctrltuser_sgadvanced ""; hasctrltuser "Has TUSER"; ctrltuserwidth "TUSER Width"; outtlastbehv "TLAST Behavior"; latencyconfig "Latency Configuration"; minimumlatency "Minimum Latency"; aclken_sgadvanced ""; aresetn_sgadvanced ""; trim_axipin_name "Display shortened port names"; aportwidth ""; bportwidth ""; ip_name ""; ip_version ""; dsptool_ready ""; ipcore_usecache ""; ipcore_useipmodelcache ""; ipcore_verbose ""; wrapper_available ""; port_translation_map ""; structural_sim ""; has_advanced_control ""; sggui_pos ""; block_type ""; block_version ""; sg_icon_stat ""; sg_mask_display ""; sg_list_contents ""; sg_blockgui_xml ""
      mask help: Xilinx Complex Multiplier 4.0
      mask init:
      | try
      |   tmp_gcb = gcb;
      |   tmp_gcbh = gcbh;
      |   if (strcmp('SysGenIndex',get_param(bdroot(tmp_gcbh),'tag')) && ~isempty(regexp(bdroot(tmp_gcb), '^xbs', 'once')))
      |     return;
      |   end;
      |   xlMungeMaskParams;
      |   block_config = 'sysgen:coregenimport_config';
      | 
      |   block_type='cmpy_v4_0';
      | 
      |   serialized_declarations = '{''aclken''=>''Bool'',''aportwidth''=>''String'',''aresetn''=>''Bool'',''atuserwidth''=>''Int'',''bportwidth''=>''String'',''btuserwidth''=>''Int'',''ctrltuserwidth''=>''Int'',''dsptool_ready''=>''Bool'',''flowcontrol''=>''String'',''hasatlast''=>''Bool'',''hasatuser''=>''Bool'',''hasbtlast''=>''Bool'',''hasbtuser''=>''Bool'',''hasctrltlast''=>''Bool'',''hasctrltuser''=>''Bool'',''ip_name''=>''String'',''ip_version''=>''String'',''ipcore_usecache''=>''Bool'',''ipcore_useipmodelcache''=>''Bool'',''ipcore_verbose''=>''Bool'',''latencyconfig''=>''String'',''minimumlatency''=>''Int'',''multtype''=>''String'',''optimizegoal''=>''String'',''outputwidth''=>''Int'',''outtlastbehv''=>''String'',''port_translation_map''=>''String'',''roundmode''=>''String'',''structural_sim''=>''Bool'',''trim_axipin_name''=>''Int'',''wrapper_available''=>''Bool'',''block_type''=>''String''}';
      |   ptable_ = xlblockprep(get_param(tmp_gcb, 'MaskWSVariables'));
      |   try
      |     xlBlockMoveCallback(tmp_gcbh);
      |   catch 
      |      clear global xl_updateicon_recursion_guard;
      |   end;
      | catch
      |   global dbgsysgen;
      |   if(~isempty(dbgsysgen) && dbgsysgen)
      |     e = regexprep(lasterr, '\n', '\nError: ');
      |     disp(['Error: While running MaskInit code on block ' tmp_gcb ': ' e]);
      |     error(e);
      |   end
      | end
      settings: CopyFcn=xlBlockMoveCallback(gcbh);  DeleteFcn=xlDestroyGui(gcbh);  ModelCloseFcn=xlDestroyGui(gcbh);  PreSaveFcn=xlBlockPreSaveCallback(gcbh);  PostSaveFcn=xlBlockPostSaveCallback(gcbh);  DestroyFcn=xlDestroyGui(gcbh);  OpenFcn=xlOpenGui(gcbh, 'cmpy_v4_0_axi_gui.xml', @xlipmagiccallback_pass_evaluate_params, @xlipmagicaction)  CloseFcn=xlDestroyGui(gcbh);  MoveFcn=xlBlockMoveCallback(gcbh);
      mask Help: eval('');xlDoc('-book','sysgen','-topic','Complex_Multiplier_4_0');
      mask StyleString: edit,checkbox,edit,checkbox,edit,edit,checkbox,edit,checkbox,edit,edit,popup(Use_Mults|Use_LUTs),edit,popup(Resources|Performance),edit,popup(Blocking|NonBlocking),edit,edit,popup(Truncate|Random_Rounding),edit,checkbox,edit,checkbox,edit,popup(Null|Pass_A_TLAST|Pass_B_TLAST|Pass_CTRL_TLAST|OR_all_TLASTs|AND_all_TLASTs),popup(Automatic|Manual),edit,edit,checkbox,edit,checkbox,checkbox,edit,edit,edit,edit,edit,edit,edit,edit,edit,edit,edit,edit,edit,edit,edit,edit,edit,edit,edit
      mask Display:
      | fprintf('','COMMENT: begin icon graphics');
      | patch([0 0 3 3 ],[154 86 86 154 ],[6.025000e-001 6.400000e-001 7.075000e-001 ]);
      | patch([0 0 3 3 ],[79 11 11 79 ],[4.350000e-001 4.600000e-001 5.050000e-001 ]);
      | patch([132 132 135 135 ],[154 6 6 154 ],[2.675000e-001 2.800000e-001 3.025000e-001 ]);
